simulink model "sim_taes_2023_att"  (R2020a)
settings: Solver=ode4  StartTime=0.0  StopTime=30.0  FixedStep=0.01  RelTol=1e-3
values from neighbouring files (symbols this model uses):
  c1_diff_sigma_bar_w = diag([12; 12; 12])    [init_taes_2023_att.m]
  c1_diff_ui = diag([25; 30; 20])    [init_taes_2023_att.m]
  c2_diff_sigma_bar_w = diag([12; 12; 12])    [init_taes_2023_att.m]
  c2_diff_ui = diag([50; 50; 10])    [init_taes_2023_att.m]
  c3_diff_sigma_bar_w = diag([15; 15; 15])    [init_taes_2023_att.m]
  c3_diff_ui = diag([15; 15; 10])    [init_taes_2023_att.m]
  cw = diag([4.0; 4.0; 4.0])    [init_taes_2023_att.m]
  dw_aa_t = 0.2 * ones(3, 5) + ( 1.0 - 0.2 ) * rand(3, 5)    [init_taes_2023_att.m]
  dw_ff_t = [ 0.4 * ones(1, 5) + ( 1.0 - 0.4 ) * rand(1, 5);                      0.4 * ones(1, 5) + ( 1.0 - 0.4 ) * rand(1, 5);                      0.2 * ones(1, 5) + ( 0.6 - 0.2 ) * rand(1, 5) ]    [init_taes_2023_att.m]
  dw_phi_t = ( - pi / 2 ) * ones(3, 5) + ( pi / 2 - ( - pi / 2 ) ) * rand(3, 5)    [init_taes_2023_att.m]
  dwci_init = zeros(3,5)    [init_taes_2023_att.m]
  h1w = diag([20.0; 20.0; 20.0])    [init_taes_2023_att.m]
  h2w = diag([35.0; 35.0; 35.0])    [init_taes_2023_att.m]
  h3w = diag([30.0; 30.0; 30.0])    [init_taes_2023_att.m]
  Ji = zeros(3,3,NF)    [init_taes_2023_att.m]
  kR = diag([40; 40; 40])    [init_taes_2023_att.m]
  kRtilt = diag([90; 90; 90])    [init_taes_2023_att.m]
  Lamd_diff_sigma_bar_w = 0.5    [init_taes_2023_att.m]
  Lamd_diff_ui = 0.5    [init_taes_2023_att.m]
  mu_d_w = 100    [init_taes_2023_att.m]
  pos0 = zeros(3, 1)    [init_taes_2023_att.m]
  PZ0 = P0(3)    [init_taes_2023_att.m]
  PZ1 = 10    [init_taes_2023_att.m]
  Qci_init = repmat([1;0;0;0],1,NF)    [init_taes_2023_att.m]
  R0 = 4    [init_taes_2023_att.m]
  R1 = 8    [init_taes_2023_att.m]
  Rci_init = zeros(3,3,NF)    [init_taes_2023_att.m]
  Ri_init = zeros(3,3,NF)    [init_taes_2023_att.m]
  Rx2 = 10    [init_taes_2023_att.m]
  Ry2 = 6    [init_taes_2023_att.m]
  Rz2 = 4    [init_taes_2023_att.m]
  T0 = 0    [init_taes_2023_att.m]
  T1 = tseq1    (= 10)    [init_taes_2023_att.m]
  T2 = tseq1 + tseq12 + tseq2    (= 30)    [init_taes_2023_att.m]
  ui_init = zeros(3,NF)    [init_taes_2023_att.m]
  vel0 = zeros(3, 1)    [init_taes_2023_att.m]
  wci_init = zeros(3,5)    [init_taes_2023_att.m]
  zeta_diff_sigma_bar_w = 0.08    [init_taes_2023_att.m]
  zeta_diff_ui = 0.08    [init_taes_2023_att.m]
undefined symbols (not defined in the file or in its folder): cal_frac_squ, p_alfaw1, p_alfaw2, q_alfaw1, q_alfaw2, Qei_init, Qeitilt_init, Qi_init, Rei_init, Reitilt_init, V_Phi_Rei_init, V_Phi_Reitilt_init, wei_init, weitilt_init, wi_init
(part 1 of 4)
settings Model: Creator=zzy  LastModifiedBy=Hershey.A
settings DataIOCC: ReturnWorkspaceOutputs=off
settings DebuggingCC: ArithmeticOperatorsInVariantConditions=warning
settings SFSimCC: SimUseLocalCustomCode=off  CustomCodeUndefinedFunction=UseInterfaceOnly
settings RTWCC: RTWUseLocalCustomCode=off

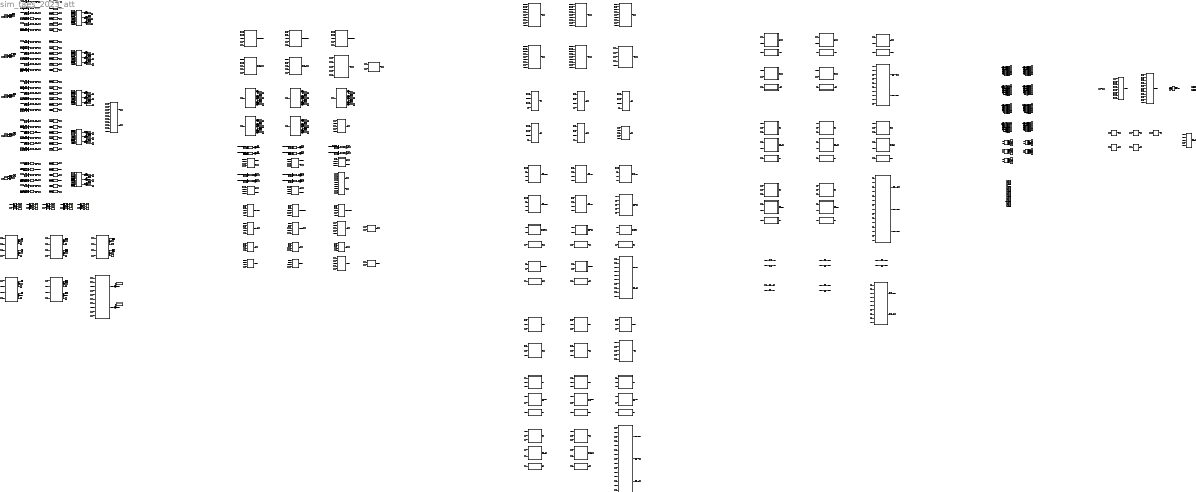
== system sim_taes_2023_att ==
  Abs{,1..29} (30 alike) : Abs
  Add{,1..2,4..6,8..10,12,14..16,18..19} (15 alike) : Sum
  Add{3,7,11,13,17} (5 alike) : Sum  Inputs=+-
  Clock : Clock
  Constant{,78,96,128,156} (5 alike) : Constant  Value=0
  Constant{1,3,5,7,9,46..47,49,65,67} (10 alike) : Constant  Value=h3w
  Constant{2,4,6,8,10,48,50,64,66,68,71,129..130,133,136,175..179} (20 alike) : Constant  Value=Ji
  Constant{51,54,59,61,63,79,82,87,89,91,97,100,105,107,109,114,119,121,123,139,142,147,149,151,157} (25 alike) : Constant
  Constant{52..53,55,62,74..75,80..81,83,90,92..93,98..99,101,108,110..111,115,122,124..125,140..141,143,150,152..153,158..159} (30 alike) : Constant  Value=3
  Constant{56,76,84,94,102,112,116,126,144,154} (10 alike) : Constant  Value=2
  Constant{57,85,103,117,145} (5 alike) : Constant  Value=c1_diff_ui
  Constant{58,86,104,118,146} (5 alike) : Constant  Value=c2_diff_ui
  Constant{60,88,106,120,148} (5 alike) : Constant  Value=c3_diff_ui
  Constant{11,13,18,23,28} (5 alike) : Constant  Value=p_alfaw1
  Constant{77,95,113,127,155} (5 alike) : Constant  Value=Lamd_diff_ui
  Constant{12,14,19,24,29} (5 alike) : Constant  Value=mu_d_w
  Constant{69,72,131,134,137} (5 alike) : Constant  Value=kR
  Constant{70,73,132,135,138} (5 alike) : Constant  Value=kRtilt
  Constant{15,20,25,30,33} (5 alike) : Constant  Value=q_alfaw1
  Constant{16,21,26,31,34} (5 alike) : Constant  Value=p_alfaw2
  Constant{160..174} (15 alike) : Constant  Value=zeta_diff_ui
  Constant{17,22,27,32,35} (5 alike) : Constant  Value=q_alfaw2
  Constant{180..184} (5 alike) : Constant  Value=cw
  Constant185 : Constant  Value=T1
  Constant186 : Constant  Value=R0
  Constant187 : Constant  Value=R1
  Constant188 : Constant  Value=T0
  Constant189 : Constant  Value=Rz2
  Constant190 : Constant  Value=Ry2
  Constant191 : Constant  Value=Rx2
  Constant192 : Constant  Value=T2
  Constant193 : Constant  Value=R0
  Constant194 : Constant  Value=R1
  Constant195 : Constant  Value=Rx2
  Constant196 : Constant  Value=Ry2
  Constant197 : Constant  Value=Rz2
  Constant198 : Constant  Value=T2
  Constant199 : Constant  Value=T1
  Constant200 : Constant  Value=PZ0
  Constant201 : Constant  Value=PZ1
  Constant{36,38,40,42,44} (5 alike) : Constant  Value=h1w
  Constant{37,39,41,43,45} (5 alike) : Constant  Value=h2w
  Constant{557,561,564,567,570} (5 alike) : Constant  Value=dw_aa_t
  Constant{558,562,565,568,572} (5 alike) : Constant  Value=dw_ff_t
  Constant{559,563,566,569,573} (5 alike) : Constant  Value=dw_phi_t
  Demux{,1..20,22..32,42..56,62..96} (82 alike) : Demux  Outputs=3
  Demux{33..37,57..61,97..101} (15 alike) : Demux
  Display{1..53,59..107} (102 alike) : Display
  Integrator{1..20} (20 alike) : Integrator  InitialCondition=zeros(3,1)
  Integrator21 : Integrator  InitialCondition=wi_init(:,1)
  Integrator22 : Integrator  InitialCondition=wi_init(:,2)
  Integrator23 : Integrator  InitialCondition=wi_init(:,3)
  Integrator24 : Integrator  InitialCondition=wi_init(:,4)
  Integrator25 : Integrator  InitialCondition=wi_init(:,5)
  Integrator26 : Integrator  InitialCondition=Qi_init(:,1)
  Integrator27 : Integrator  InitialCondition=Qi_init(:,2)
  Integrator28 : Integrator  InitialCondition=Qi_init(:,3)
  Integrator29 : Integrator  InitialCondition=Qi_init(:,4)
  Integrator30 : Integrator  InitialCondition=Qi_init(:,5)
  Integrator31 : Integrator  InitialCondition=Qei_init(:,1)
  Integrator32 : Integrator  InitialCondition=Qei_init(:,2)
  Integrator33 : Integrator  InitialCondition=Qei_init(:,3)
  Integrator34 : Integrator  InitialCondition=Qei_init(:,4)
  Integrator35 : Integrator  InitialCondition=Qei_init(:,5)
  Integrator36 : Integrator  InitialCondition=Qeitilt_init(:,1)
  Integrator37 : Integrator  InitialCondition=Qeitilt_init(:,2)
  Integrator38 : Integrator  InitialCondition=Qeitilt_init(:,3)
  Integrator39 : Integrator  InitialCondition=Qeitilt_init(:,4)
  Integrator40 : Integrator  InitialCondition=Qeitilt_init(:,5)
  Integrator41 : Integrator  InitialCondition=V_Phi_Reitilt_init(:,1)
  Integrator42 : Integrator  InitialCondition=V_Phi_Rei_init(:,2)
  Integrator43 : Integrator  InitialCondition=V_Phi_Reitilt_init(:,2)
  Integrator44 : Integrator  InitialCondition=V_Phi_Rei_init(:,3)
  Integrator45 : Integrator  InitialCondition=V_Phi_Rei_init(:,1)
  Integrator46 : Integrator  InitialCondition=V_Phi_Reitilt_init(:,3)
  Integrator47 : Integrator  InitialCondition=V_Phi_Rei_init(:,4)
  Integrator48 : Integrator  InitialCondition=V_Phi_Reitilt_init(:,4)
  Integrator49 : Integrator  InitialCondition=V_Phi_Rei_init(:,5)
  Integrator50 : Integrator  InitialCondition=V_Phi_Reitilt_init(:,5)
  Interpreted MATLAB Function{,1..39} (40 alike) : MATLABFcn  MATLABFcn=cal_frac_squ(u(1:3),u(4),u(5))
  Memory : Memory  InitialCondition=ui_init
  Memory10 : Memory  InitialCondition=Qeitilt_init
  Memory11 : Memory  InitialCondition=Reitilt_init
  Memory12 : Memory  InitialCondition=V_Phi_Rei_init
  Memory13 : Memory  InitialCondition=V_Phi_Reitilt_init
  Memory14 : Memory  InitialCondition=wci_init
  Memory15 : Memory  InitialCondition=dwci_init
  Memory16 : Memory  InitialCondition=Qci_init
  Memory17 : Memory  InitialCondition=Rci_init
  Memory3 : Memory  InitialCondition=Qi_init
  Memory4 : Memory  InitialCondition=Ri_init
  Memory5 : Memory  InitialCondition=wi_init
  Memory6 : Memory  InitialCondition=wei_init
  Memory7 : Memory  InitialCondition=Qei_init
  Memory8 : Memory  InitialCondition=Rei_init
  Memory9 : Memory  InitialCondition=weitilt_init
  Mux{,41..69} (30 alike) : Mux  Inputs=2
  Mux{1..40} (40 alike) : Mux  Inputs=3
  Product{,1..9} (10 alike) : Product
  Qei dynam agent 1 : MATLAB Function  TreatAsAtomicUnit=on
  Qei dynam agent 2 : MATLAB Function  TreatAsAtomicUnit=on
  Qei dynam agent 3 : MATLAB Function  TreatAsAtomicUnit=on
  Qei dynam agent 4 : MATLAB Function  TreatAsAtomicUnit=on
  Qei dynam agent 5 : MATLAB Function  TreatAsAtomicUnit=on
  Qeitilt dynam agent 1 : MATLAB Function  TreatAsAtomicUnit=on
  Qeitilt dynam agent 2 : MATLAB Function  TreatAsAtomicUnit=on
  Qeitilt dynam agent 3 : MATLAB Function  TreatAsAtomicUnit=on
  Qeitilt dynam agent 4 : MATLAB Function  TreatAsAtomicUnit=on
  Qeitilt dynam agent 5 : MATLAB Function  TreatAsAtomicUnit=on
  Qi dynam agent 1 : MATLAB Function  TreatAsAtomicUnit=on
  Qi dynam agent 2 : MATLAB Function  TreatAsAtomicUnit=on
  Qi dynam agent 3 : MATLAB Function  TreatAsAtomicUnit=on
  Qi dynam agent 4 : MATLAB Function  TreatAsAtomicUnit=on
  Qi dynam agent 5 : MATLAB Function  TreatAsAtomicUnit=on
  Scope{,3..11,45..49} (15 alike) : Scope  NumInputPorts=4
  Scope{1..2,12..44} (35 alike) : Scope  NumInputPorts=3
  Step : Step  Time=T1+0.01  SampleTime=0
  To Workspace : ToWorkspace  VariableName=wci  SampleTime=-1
  To Workspace1 : ToWorkspace  VariableName=V_Phi_Rei  SampleTime=-1
  To Workspace10 : ToWorkspace  VariableName=dwi_tilt  SampleTime=-1
  To Workspace11 : ToWorkspace  VariableName=Qci  SampleTime=-1
  To Workspace12 : ToWorkspace  VariableName=sigma_bar_w_hat  SampleTime=-1
  To Workspace13 : ToWorkspace  VariableName=wei  SampleTime=-1
  To Workspace14 : ToWorkspace  VariableName=sigma_w  SampleTime=-1
  To Workspace15 : ToWorkspace  VariableName=sigma_bar_w  SampleTime=-1
  To Workspace16 : ToWorkspace  VariableName=weitilt  SampleTime=-1
  To Workspace19 : ToWorkspace  VariableName=Qei  SampleTime=-1
  To Workspace2 : ToWorkspace  VariableName=wi  SampleTime=-1
  To Workspace20 : ToWorkspace  VariableName=Qi  SampleTime=-1
  To Workspace6 : ToWorkspace  VariableName=V_Phi_Reitilt  SampleTime=-1
  To Workspace7 : ToWorkspace  VariableName=Qeitilt  SampleTime=-1
  To Workspace8 : ToWorkspace  VariableName=dwi  SampleTime=-1
  To Workspace9 : ToWorkspace  VariableName=dwi_hat  SampleTime=-1
  cal Qci agent 1 : MATLAB Function  TreatAsAtomicUnit=on
  cal Qci agent 2 : MATLAB Function  TreatAsAtomicUnit=on
  cal Qci agent 3 : MATLAB Function  TreatAsAtomicUnit=on
  cal Qci agent 4 : MATLAB Function  TreatAsAtomicUnit=on
  cal Qci agent 5 : MATLAB Function  TreatAsAtomicUnit=on
  cal Rci agent 1 : MATLAB Function  TreatAsAtomicUnit=on
  cal Rci agent 2 : MATLAB Function  TreatAsAtomicUnit=on
  cal Rci agent 3 : MATLAB Function  TreatAsAtomicUnit=on
  cal Rci agent 4 : MATLAB Function  TreatAsAtomicUnit=on
  cal Rci agent 5 : MATLAB Function  TreatAsAtomicUnit=on
  cal Rei agent 1 : MATLAB Function  TreatAsAtomicUnit=on
  cal Rei agent 2 : MATLAB Function  TreatAsAtomicUnit=on
  cal Rei agent 3 : MATLAB Function  TreatAsAtomicUnit=on
  cal Rei agent 4 : MATLAB Function  TreatAsAtomicUnit=on
  cal Rei agent 5 : MATLAB Function  TreatAsAtomicUnit=on
  cal Reitilt agent 1 : MATLAB Function  TreatAsAtomicUnit=on
  cal Reitilt agent 2 : MATLAB Function  TreatAsAtomicUnit=on
  cal Reitilt agent 3 : MATLAB Function  TreatAsAtomicUnit=on
  cal Reitilt agent 4 : MATLAB Function  TreatAsAtomicUnit=on
  cal Reitilt agent 5 : MATLAB Function  TreatAsAtomicUnit=on
  cal Ri agent 1 : MATLAB Function  TreatAsAtomicUnit=on
  cal Ri agent 2 : MATLAB Function  TreatAsAtomicUnit=on
  cal Ri agent 3 : MATLAB Function  TreatAsAtomicUnit=on
  cal Ri agent 4 : MATLAB Function  TreatAsAtomicUnit=on
  cal Ri agent 5 : MATLAB Function  TreatAsAtomicUnit=on
  cal abs 21 : MATLAB Function  TreatAsAtomicUnit=on
  cal abs 22 : MATLAB Function  TreatAsAtomicUnit=on
  cal abs 23 : MATLAB Function  TreatAsAtomicUnit=on
  cal abs 24 : MATLAB Function  TreatAsAtomicUnit=on
  cal abs 25 : MATLAB Function  TreatAsAtomicUnit=on
  cal abs 26 : MATLAB Function  TreatAsAtomicUnit=on
  cal abs 27 : MATLAB Function  TreatAsAtomicUnit=on
  cal abs 28 : MATLAB Function  TreatAsAtomicUnit=on
  cal abs 29 : MATLAB Function  TreatAsAtomicUnit=on
  cal abs 30 : MATLAB Function  TreatAsAtomicUnit=on
  cal combine sigma_bar_w_tilt : MATLAB Function  TreatAsAtomicUnit=on
  cal d_sigma_w agent 1 : MATLAB Function  TreatAsAtomicUnit=on
  cal d_sigma_w agent 2 : MATLAB Function  TreatAsAtomicUnit=on
  cal d_sigma_w agent 3 : MATLAB Function  TreatAsAtomicUnit=on
  cal d_sigma_w agent 4 : MATLAB Function  TreatAsAtomicUnit=on
  cal d_sigma_w agent 5 : MATLAB Function  TreatAsAtomicUnit=on
  cal d_theta_hat : MATLAB Function  TreatAsAtomicUnit=on
  cal d_theta_hat1 : MATLAB Function  TreatAsAtomicUnit=on
  cal d_theta_hat2 : MATLAB Function  TreatAsAtomicUnit=on
  cal d_theta_hat3 : MATLAB Function  TreatAsAtomicUnit=on
  cal d_theta_hat4 : MATLAB Function  TreatAsAtomicUnit=on
  cal differentiator d_sigma_bar_w_hat agent 1 : Subsystem
  cal differentiator d_sigma_bar_w_hat agent 2 : Subsystem
  cal differentiator d_sigma_bar_w_hat agent 3 : Subsystem
  cal differentiator d_sigma_bar_w_hat agent 4 : Subsystem
  cal differentiator d_sigma_bar_w_hat agent 5 : Subsystem
  cal dw_hat agent 1 : MATLAB Function  TreatAsAtomicUnit=on
  cal dw_hat agent 2 : MATLAB Function  TreatAsAtomicUnit=on
  cal dw_hat agent 3 : MATLAB Function  TreatAsAtomicUnit=on
  cal dw_hat agent 4 : MATLAB Function  TreatAsAtomicUnit=on
  cal dw_hat agent 5 : MATLAB Function  TreatAsAtomicUnit=on
  cal error dw_tilt : MATLAB Function  TreatAsAtomicUnit=on
  cal sig : MATLAB Function  TreatAsAtomicUnit=on
  cal sig1 : MATLAB Function  TreatAsAtomicUnit=on
  cal sig10 : MATLAB Function  TreatAsAtomicUnit=on
  cal sig11 : MATLAB Function  TreatAsAtomicUnit=on
  cal sig12 : MATLAB Function  TreatAsAtomicUnit=on
  cal sig13 : MATLAB Function  TreatAsAtomicUnit=on
  cal sig14 : MATLAB Function  TreatAsAtomicUnit=on
  cal sig15 : MATLAB Function  TreatAsAtomicUnit=on
  cal sig16 : MATLAB Function  TreatAsAtomicUnit=on
  cal sig17 : MATLAB Function  TreatAsAtomicUnit=on
  cal sig18 : MATLAB Function  TreatAsAtomicUnit=on
  cal sig19 : MATLAB Function  TreatAsAtomicUnit=on
  cal sig2 : MATLAB Function  TreatAsAtomicUnit=on
  cal sig20 : MATLAB Function  TreatAsAtomicUnit=on
  cal sig21 : MATLAB Function  TreatAsAtomicUnit=on
  cal sig22 : MATLAB Function  TreatAsAtomicUnit=on
  cal sig23 : MATLAB Function  TreatAsAtomicUnit=on
  cal sig24 : MATLAB Function  TreatAsAtomicUnit=on
  cal sig25 : MATLAB Function  TreatAsAtomicUnit=on
  cal sig26 : MATLAB Function  TreatAsAtomicUnit=on
  cal sig27 : MATLAB Function  TreatAsAtomicUnit=on
  cal sig28 : MATLAB Function  TreatAsAtomicUnit=on
  cal sig29 : MATLAB Function  TreatAsAtomicUnit=on
  cal sig3 : MATLAB Function  TreatAsAtomicUnit=on
  cal sig4 : MATLAB Function  TreatAsAtomicUnit=on
  cal sig5 : MATLAB Function  TreatAsAtomicUnit=on
  cal sig6 : MATLAB Function  TreatAsAtomicUnit=on
  cal sig7 : MATLAB Function  TreatAsAtomicUnit=on
  cal sig8 : MATLAB Function  TreatAsAtomicUnit=on
  cal sig9 : MATLAB Function  TreatAsAtomicUnit=on
  cal sigma_bar_w_hat agent 1 : MATLAB Function  TreatAsAtomicUnit=on
  cal sigma_bar_w_hat agent 2 : MATLAB Function  TreatAsAtomicUnit=on
  cal sigma_bar_w_hat agent 3 : MATLAB Function  TreatAsAtomicUnit=on
  cal sigma_bar_w_hat agent 4 : MATLAB Function  TreatAsAtomicUnit=on
  cal sigma_bar_w_hat agent 5 : MATLAB Function  TreatAsAtomicUnit=on
  cal sigma_w_bar : MATLAB Function  TreatAsAtomicUnit=on
  cal taui agent 1 : MATLAB Function  TreatAsAtomicUnit=on
  cal taui agent 2 : MATLAB Function  TreatAsAtomicUnit=on
  cal taui agent 3 : MATLAB Function  TreatAsAtomicUnit=on
  cal taui agent 4 : MATLAB Function  TreatAsAtomicUnit=on
  cal taui agent 5 : MATLAB Function  TreatAsAtomicUnit=on
  cal theta_sigma_bar_w_tilt agent 1 : MATLAB Function  TreatAsAtomicUnit=on
  cal theta_sigma_bar_w_tilt agent 2 : MATLAB Function  TreatAsAtomicUnit=on
  cal theta_sigma_bar_w_tilt agent 3 : MATLAB Function  TreatAsAtomicUnit=on
  cal theta_sigma_bar_w_tilt agent 4 : MATLAB Function  TreatAsAtomicUnit=on
  cal theta_sigma_bar_w_tilt agent 5 : MATLAB Function  TreatAsAtomicUnit=on
  cal wbarei agent 1 : MATLAB Function  TreatAsAtomicUnit=on
  cal wbarei agent 2 : MATLAB Function  TreatAsAtomicUnit=on
  cal wbarei agent 3 : MATLAB Function  TreatAsAtomicUnit=on
  cal wbarei agent 4 : MATLAB Function  TreatAsAtomicUnit=on
  cal wbarei agent 5 : MATLAB Function  TreatAsAtomicUnit=on
  cal wci dwci agent 1 : MATLAB Function  TreatAsAtomicUnit=on
  cal wci dwci agent 2 : MATLAB Function  TreatAsAtomicUnit=on
  cal wci dwci agent 3 : MATLAB Function  TreatAsAtomicUnit=on
  cal wci dwci agent 4 : MATLAB Function  TreatAsAtomicUnit=on
  cal wci dwci agent 5 : MATLAB Function  TreatAsAtomicUnit=on
  cal wei agent 1 : MATLAB Function  TreatAsAtomicUnit=on
  cal wei agent 2 : MATLAB Function  TreatAsAtomicUnit=on
  cal wei agent 3 : MATLAB Function  TreatAsAtomicUnit=on
  cal wei agent 4 : MATLAB Function  TreatAsAtomicUnit=on
  cal wei agent 5 : MATLAB Function  TreatAsAtomicUnit=on
  cal weitilt agent 1 : MATLAB Function  TreatAsAtomicUnit=on
  cal weitilt agent 2 : MATLAB Function  TreatAsAtomicUnit=on
  cal weitilt agent 3 : MATLAB Function  TreatAsAtomicUnit=on
  cal weitilt agent 4 : MATLAB Function  TreatAsAtomicUnit=on
  cal weitilt agent 5 : MATLAB Function  TreatAsAtomicUnit=on
  choose ksi_est_err 21 : MATLAB Function  TreatAsAtomicUnit=on
  choose ksi_est_err 22 : MATLAB Function  TreatAsAtomicUnit=on
  choose ksi_est_err 23 : MATLAB Function  TreatAsAtomicUnit=on
  choose ksi_est_err 24 : MATLAB Function  TreatAsAtomicUnit=on
  choose ksi_est_err 25 : MATLAB Function  TreatAsAtomicUnit=on
  choose ksi_est_err 26 : MATLAB Function  TreatAsAtomicUnit=on
  choose ksi_est_err 27 : MATLAB Function  TreatAsAtomicUnit=on
  choose ksi_est_err 28 : MATLAB Function  TreatAsAtomicUnit=on
  choose ksi_est_err 29 : MATLAB Function  TreatAsAtomicUnit=on
  choose ksi_est_err 30 : MATLAB Function  TreatAsAtomicUnit=on
  choose ui agent 1 : MATLAB Function  TreatAsAtomicUnit=on
  choose ui agent 2 : MATLAB Function  TreatAsAtomicUnit=on
  choose ui agent 3 : MATLAB Function  TreatAsAtomicUnit=on
  choose ui agent 4 : MATLAB Function  TreatAsAtomicUnit=on
  choose ui agent 5 : MATLAB Function  TreatAsAtomicUnit=on
  combine Qci Rci : MATLAB Function  TreatAsAtomicUnit=on
  combine Qci Rci1 : MATLAB Function  TreatAsAtomicUnit=on
  combine Qi Ri : MATLAB Function  TreatAsAtomicUnit=on
  combine d_sigma_bar_v_est : MATLAB Function  TreatAsAtomicUnit=on
  combine duihat d2uihat : MATLAB Function  TreatAsAtomicUnit=on
  combine dw_hat : MATLAB Function  TreatAsAtomicUnit=on
  combine dwi : MATLAB Function  TreatAsAtomicUnit=on
  combine norminal formation control input : MATLAB Function  TreatAsAtomicUnit=on
  combine sigma_bar_w_hat : MATLAB Function  TreatAsAtomicUnit=on
  combine sigma_w : MATLAB Function  TreatAsAtomicUnit=on
  combine tau : MATLAB Function  TreatAsAtomicUnit=on
  combine tau1 : MATLAB Function  TreatAsAtomicUnit=on
  combine theta_sigma_bar_w_tilt : MATLAB Function  TreatAsAtomicUnit=on
  combine wbarei : MATLAB Function  TreatAsAtomicUnit=on
  combine wci dwci : MATLAB Function  TreatAsAtomicUnit=on
  combine wei Qei Rei : MATLAB Function  TreatAsAtomicUnit=on
  combine weitilt Qeitilt Reitilt : MATLAB Function  TreatAsAtomicUnit=on
  control input generator agent 1 : MATLAB Function  TreatAsAtomicUnit=on
  control input generator agent 2 : MATLAB Function  TreatAsAtomicUnit=on
  control input generator agent 3 : MATLAB Function  TreatAsAtomicUnit=on
  control input generator agent 4 : MATLAB Function  TreatAsAtomicUnit=on
  control input generator agent 5 : MATLAB Function  TreatAsAtomicUnit=on
  d2_sigma_bar_w_est_{1..5} (5 alike) : Scope  NumInputPorts=3
  d2_ui_hat_node_{1..5} (5 alike) : Scope  NumInputPorts=3
  d_sigma_bar_w_est_{1..5} (5 alike) : Scope  NumInputPorts=3
  d_ui_hat_node_{1..5} (5 alike) : Scope  NumInputPorts=3
  depart Qc1 : MATLAB Function  TreatAsAtomicUnit=on
  depart Qc2 : MATLAB Function  TreatAsAtomicUnit=on
  depart Qc3 : MATLAB Function  TreatAsAtomicUnit=on
  depart Qc4 : MATLAB Function  TreatAsAtomicUnit=on
  depart Qc5 : MATLAB Function  TreatAsAtomicUnit=on
  depart Qe1 : MATLAB Function  TreatAsAtomicUnit=on
  depart Qe1tilt : MATLAB Function  TreatAsAtomicUnit=on
  depart Qe2 : MATLAB Function  TreatAsAtomicUnit=on
  depart Qe2tilt : MATLAB Function  TreatAsAtomicUnit=on
  depart Qe3 : MATLAB Function  TreatAsAtomicUnit=on
  depart Qe3tilt : MATLAB Function  TreatAsAtomicUnit=on
  depart Qe4 : MATLAB Function  TreatAsAtomicUnit=on
  depart Qe4tilt : MATLAB Function  TreatAsAtomicUnit=on
  depart Qe5 : MATLAB Function  TreatAsAtomicUnit=on
  depart Qe5tilt : MATLAB Function  TreatAsAtomicUnit=on
  depart V_Phi_Re1 : MATLAB Function  TreatAsAtomicUnit=on
  depart V_Phi_Re1tilt : MATLAB Function  TreatAsAtomicUnit=on
  depart V_Phi_Re2 : MATLAB Function  TreatAsAtomicUnit=on
  depart V_Phi_Re2tilt : MATLAB Function  TreatAsAtomicUnit=on
  depart V_Phi_Re3 : MATLAB Function  TreatAsAtomicUnit=on
  depart V_Phi_Re3tilt : MATLAB Function  TreatAsAtomicUnit=on
  depart V_Phi_Re4 : MATLAB Function  TreatAsAtomicUnit=on
  depart V_Phi_Re4tilt : MATLAB Function  TreatAsAtomicUnit=on
  depart V_Phi_Re5 : MATLAB Function  TreatAsAtomicUnit=on
  depart V_Phi_Re5tilt : MATLAB Function  TreatAsAtomicUnit=on
  depart dw1 dw_hat_1 : MATLAB Function  TreatAsAtomicUnit=on
  depart dw2 dw_hat_2 : MATLAB Function  TreatAsAtomicUnit=on
  depart dw3 dw_hat_3 : MATLAB Function  TreatAsAtomicUnit=on
  depart dw4 dw_hat_1 : MATLAB Function  TreatAsAtomicUnit=on
  depart dw4 dw_hat_4 : MATLAB Function  TreatAsAtomicUnit=on
  depart wc1 : MATLAB Function  TreatAsAtomicUnit=on
  depart wc2 : MATLAB Function  TreatAsAtomicUnit=on
  depart wc3 : MATLAB Function  TreatAsAtomicUnit=on
  depart wc4 : MATLAB Function  TreatAsAtomicUnit=on
  depart wc5 : MATLAB Function  TreatAsAtomicUnit=on
  depart we1 : MATLAB Function  TreatAsAtomicUnit=on
  depart we1tilt : MATLAB Function  TreatAsAtomicUnit=on
  depart we2 : MATLAB Function  TreatAsAtomicUnit=on
  depart we2tilt : MATLAB Function  TreatAsAtomicUnit=on
  depart we3 : MATLAB Function  TreatAsAtomicUnit=on
  depart we3tilt : MATLAB Function  TreatAsAtomicUnit=on
  depart we4 : MATLAB Function  TreatAsAtomicUnit=on
  depart we4tilt : MATLAB Function  TreatAsAtomicUnit=on
  depart we5 : MATLAB Function  TreatAsAtomicUnit=on
  depart we5tilt : MATLAB Function  TreatAsAtomicUnit=on
  dwci_node_{1..5} (5 alike) : Scope  NumInputPorts=3
  eta_0 : Scope  NumInputPorts=3
  generate angular rate disturbance agent 1 : MATLAB Function  TreatAsAtomicUnit=on
  generate angular rate disturbance agent 2 : MATLAB Function  TreatAsAtomicUnit=on
  generate angular rate disturbance agent 3 : MATLAB Function  TreatAsAtomicUnit=on
  generate angular rate disturbance agent 4 : MATLAB Function  TreatAsAtomicUnit=on
  generate angular rate disturbance agent 5 : MATLAB Function  TreatAsAtomicUnit=on
  ksi_0 : Scope  NumInputPorts=3
  leader control input : MATLAB Function  TreatAsAtomicUnit=on
  leader eta0 Integrator : Integrator  ExternalReset=rising  InitialConditionSource=external  InitialCondition=vel0
  leader ksi0 Integrator : Integrator  InitialCondition=pos0
  process velocity : MATLAB Function  TreatAsAtomicUnit=on
  sigma_bar_w_hat Integrator {1..5} (5 alike) : Integrator  InitialCondition=zeros(3,1)
  trans to column1 : MATLAB Function  TreatAsAtomicUnit=on
  trans to column10 : MATLAB Function  TreatAsAtomicUnit=on
  trans to column11 : MATLAB Function  TreatAsAtomicUnit=on
  trans to column12 : MATLAB Function  TreatAsAtomicUnit=on
  trans to column13 : MATLAB Function  TreatAsAtomicUnit=on
  trans to column14 : MATLAB Function  TreatAsAtomicUnit=on
  trans to column15 : MATLAB Function  TreatAsAtomicUnit=on
  trans to column16 : MATLAB Function  TreatAsAtomicUnit=on
  trans to column17 : MATLAB Function  TreatAsAtomicUnit=on
  trans to column18 : MATLAB Function  TreatAsAtomicUnit=on
  trans to column19 : MATLAB Function  TreatAsAtomicUnit=on
  trans to column2 : MATLAB Function  TreatAsAtomicUnit=on
  trans to column20 : MATLAB Function  TreatAsAtomicUnit=on
  trans to column21 : MATLAB Function  TreatAsAtomicUnit=on
  trans to column22 : MATLAB Function  TreatAsAtomicUnit=on
  trans to column23 : MATLAB Function  TreatAsAtomicUnit=on
  trans to column24 : MATLAB Function  TreatAsAtomicUnit=on
  trans to column25 : MATLAB Function  TreatAsAtomicUnit=on
  trans to column26 : MATLAB Function  TreatAsAtomicUnit=on
  trans to column27 : MATLAB Function  TreatAsAtomicUnit=on
  trans to column28 : MATLAB Function  TreatAsAtomicUnit=on
  trans to column29 : MATLAB Function  TreatAsAtomicUnit=on
  trans to column3 : MATLAB Function  TreatAsAtomicUnit=on
  trans to column30 : MATLAB Function  TreatAsAtomicUnit=on
  trans to column31 : MATLAB Function  TreatAsAtomicUnit=on
  trans to column32 : MATLAB Function  TreatAsAtomicUnit=on
  trans to column33 : MATLAB Function  TreatAsAtomicUnit=on
  trans to column34 : MATLAB Function  TreatAsAtomicUnit=on
  trans to column35 : MATLAB Function  TreatAsAtomicUnit=on
  trans to column36 : MATLAB Function  TreatAsAtomicUnit=on
  trans to column37 : MATLAB Function  TreatAsAtomicUnit=on
  trans to column38 : MATLAB Function  TreatAsAtomicUnit=on
  trans to column39 : MATLAB Function  TreatAsAtomicUnit=on
  trans to column4 : MATLAB Function  TreatAsAtomicUnit=on
  trans to column40 : MATLAB Function  TreatAsAtomicUnit=on
  trans to column5 : MATLAB Function  TreatAsAtomicUnit=on
  trans to column6 : MATLAB Function  TreatAsAtomicUnit=on
  trans to column7 : MATLAB Function  TreatAsAtomicUnit=on
  trans to column8 : MATLAB Function  TreatAsAtomicUnit=on
  trans to column9 : MATLAB Function  TreatAsAtomicUnit=on
  ui_tilt_node_{1..5} (5 alike) : Scope  NumInputPorts=3
  wci_node_{1..5} (5 alike) : Scope  NumInputPorts=3
  wi dynam agent 1 : MATLAB Function  TreatAsAtomicUnit=on
  wi dynam agent 2 : MATLAB Function  TreatAsAtomicUnit=on
  wi dynam agent 3 : MATLAB Function  TreatAsAtomicUnit=on
  wi dynam agent 4 : MATLAB Function  TreatAsAtomicUnit=on
  wi dynam agent 5 : MATLAB Function  TreatAsAtomicUnit=on
  wires:
  [d_ui_hat_node_1] -> cal d_theta_hat/11(dui_hat)
  [ui_sig_3_node_1] -> cal d_theta_hat/7(ui_sig_3)
  cal d_theta_hat/2(d_dui_hat) -> Integrator3/1
  Constant63/1 -> Mux8/2
  Mux10/1 -> Interpreted MATLAB Function9/1
  cal sig5/1(z) -> [ui_sig_5_node_1]
  Interpreted MATLAB Function8/1 -> trans to column8/1(x)
  Interpreted MATLAB Function9/1 -> trans to column9/1(x)
  [ui_squ_3_node_1] -> cal sig2/1(x)
  Constant163/1 -> Product1/2
  [ui_squ_6_node_1] -> cal sig3/1(x)
  [ui_sig_6_node_1] -> cal d_theta_hat/10(ui_sig_6)
  cal d_theta_hat/3(d_d2ui_hat) -> Integrator4/1
  trans to column8/1(y) -> [ui_squ_4_node_1]
  [ui_tilt_node_1] -> cal sig1/2(y)
  [ui_sig_2_node_1] -> cal d_theta_hat/6(ui_sig_2)
  Abs/1 -> Mux7/1
  Constant56/1 -> Mux11/2
  [d2_ui_hat_node_1] -> cal d_theta_hat/12(d2ui_hat)
  cal sig3/1(z) -> [ui_sig_6_node_1]
  Interpreted MATLAB Function7/1 -> trans to column7/1(x)
  Interpreted MATLAB Function/1 -> trans to column6/1(x)
  cal sig4/1(z) -> [ui_sig_4_node_1]
  Product1/1 -> Add2/2
  [ui_tilt_node_1] -> cal sig5/2(y)
  trans to column10/1(y) -> [ui_squ_5_node_1]
  [ui_tilt_node_1] -> cal sig/2(y)
  Interpreted MATLAB Function10/1 -> trans to column10/1(x)
  Mux11/1 -> Interpreted MATLAB Function10/1
  Abs5/1 -> Mux11/1
  Abs3/1 -> Mux9/1
  Constant53/1 -> Add2/1
  Constant/1 -> Mux7/2
  Constant162/1 -> Product/2
  Constant54/1 -> Product1/1
  Constant55/1 -> Mux11/3
  [ui_tilt_node_1] -> Abs4/1
  [ui_sig_4_node_1] -> cal d_theta_hat/8(ui_sig_4)
  [ui_sig_1_node_1] -> cal d_theta_hat/5(ui_sig_1)
  [ui_squ_5_node_1] -> cal sig5/1(x)
  Constant59/1 -> Add/1
  Constant61/1 -> Mux6/3
  Mux7/1 -> Interpreted MATLAB Function/1
  Mux8/1 -> Interpreted MATLAB Function7/1
  Constant161/1 -> Add/2
  [ui_tilt_node_1] -> Abs2/1
  [ui_tilt_node_1] -> Abs1/1
  [ui_tilt_node_1] -> Abs5/1
  Mux6/1 -> Interpreted MATLAB Function6/1
  Interpreted MATLAB Function6/1 -> trans to column5/1(x)
  Add/1 -> Mux6/2
  [ui_squ_4_node_1] -> cal sig4/1(x)
  trans to column9/1(y) -> [ui_squ_6_node_1]
  trans to column7/1(y) -> [ui_squ_3_node_1]
  [ui_tilt_node_1] -> cal sig4/2(y)
  [ui_tilt_node_1] -> cal sig3/2(y)
  Product/1 -> Add1/2
  Constant51/1 -> Mux7/3
  Constant75/1 -> Add1/1
  [ui_tilt_node_1] -> Abs/1
  [ui_tilt_node_1] -> Abs3/1
  Mux9/1 -> Interpreted MATLAB Function8/1
  Abs2/1 -> Mux8/1
  Constant62/1 -> Mux8/3
  trans to column5/1(y) -> [ui_squ_2_node_1]
  cal sig1/1(z) -> [ui_sig_2_node_1]
  Constant52/1 -> Mux10/3
  cal sig/1(z) -> [ui_sig_1_node_1]
  Abs4/1 -> Mux10/1
  cal sig2/1(z) -> [ui_sig_3_node_1]
  Abs1/1 -> Mux6/1
  Constant74/1 -> Mux9/3
  Add2/1 -> Mux10/2
  [ui_sig_5_node_1] -> cal d_theta_hat/9(ui_sig_5)
  Add1/1 -> Mux9/2
  Constant76/1 -> Product/1
  [ui_tilt_node_1] -> cal sig2/2(y)
  [ui_squ_2_node_1] -> cal sig1/1(x)
  [ui_squ_1_node_1] -> cal sig/1(x)
  trans to column6/1(y) -> [ui_squ_1_node_1]
  Constant57/1 -> cal d_theta_hat/1(c1)
  Constant58/1 -> cal d_theta_hat/2(c2)
  Constant60/1 -> cal d_theta_hat/3(c3)
  Constant77/1 -> cal d_theta_hat/4(chi_t)
  Integrator4/1 -> Display24/1, Demux12/1, [d2_ui_hat_node_1]
  cal d_theta_hat/1(d_ui_hat) -> Integrator2/1
  Integrator3/1 -> Demux8/1, Display23/1, [d_ui_hat_node_1]
  Integrator2/1 -> Display22/1, [ui_hat_node_1]
  [ui_hat_node_1] -> Add3/1
  Add3/1 -> Demux2/1, [ui_tilt_node_1]
  [ui_vec] -> choose ui agent 1/1(x)
  choose ui agent 1/1(y) -> Add3/2
  [ui_squ_1_node_2] -> cal sig6/1(x)
  [ui_squ_2_node_2] -> cal sig7/1(x)
  [ui_tilt_node_2] -> cal sig8/2(y)
  Constant94/1 -> Product2/1
  Constant95/1 -> cal d_theta_hat1/4(chi_t)
  Add7/1 -> Demux3/1, [ui_tilt_node_2]
  [ui_hat_node_2] -> Add7/1
  [ui_sig_5_node_2] -> cal d_theta_hat1/9(ui_sig_5)
  Add6/1 -> Mux12/2
  Add5/1 -> Mux17/2
  Constant92/1 -> Mux17/3
  Constant80/1 -> Mux12/3
  cal sig6/1(z) -> [ui_sig_1_node_2]
  trans to column12/1(y) -> [ui_squ_2_node_2]
  cal sig7/1(z) -> [ui_sig_2_node_2]
  cal sig8/1(z) -> [ui_sig_3_node_2]
  Abs7/1 -> Mux14/1
  Abs10/1 -> Mux12/1
  Constant90/1 -> Mux16/3
  [ui_tilt_node_2] -> Abs9/1
  Mux17/1 -> Interpreted MATLAB Function15/1
  choose ui agent 2/1(y) -> Add7/2
  Abs8/1 -> Mux16/1
  Product2/1 -> Add5/2
  [ui_tilt_node_2] -> Abs6/1
  Constant93/1 -> Add5/1
  [ui_tilt_node_2] -> cal sig10/2(y)
  Constant79/1 -> Mux15/3
  trans to column16/1(y) -> [ui_squ_6_node_2]
  Constant88/1 -> cal d_theta_hat1/3(c3)
  Constant85/1 -> cal d_theta_hat1/1(c1)
  Integrator1/1 -> Display25/1, [ui_hat_node_2]
  Integrator6/1 -> Display27/1, Demux13/1, [d2_ui_hat_node_2]
  trans to column15/1(y) -> [ui_squ_4_node_2]
  [ui_sig_6_node_2] -> cal d_theta_hat1/10(ui_sig_6)
  [ui_squ_6_node_2] -> cal sig9/1(x)
  Constant91/1 -> Mux16/2
  [ui_squ_4_node_2] -> cal sig10/1(x)
  [d_ui_hat_node_2] -> cal d_theta_hat1/11(dui_hat)
  Mux14/1 -> Interpreted MATLAB Function13/1
  [ui_tilt_node_2] -> cal sig9/2(y)
  Constant160/1 -> Add4/2
  Constant87/1 -> Add4/1
  Mux12/1 -> Interpreted MATLAB Function16/1
  [ui_squ_5_node_2] -> cal sig11/1(x)
  [ui_sig_1_node_2] -> cal d_theta_hat1/5(ui_sig_1)
  [ui_tilt_node_2] -> Abs8/1
  [ui_sig_4_node_2] -> cal d_theta_hat1/8(ui_sig_4)
  [ui_tilt_node_2] -> Abs10/1
  cal d_theta_hat1/2(d_dui_hat) -> Integrator5/1
  Constant89/1 -> Mux14/3
  Constant83/1 -> Mux13/3
  Constant82/1 -> Product3/1
  Abs9/1 -> Mux17/1
  Interpreted MATLAB Function11/1 -> trans to column13/1(x)
  Mux16/1 -> Interpreted MATLAB Function14/1
  trans to column13/1(y) -> [ui_squ_1_node_2]
  Interpreted MATLAB Function16/1 -> trans to column16/1(x)
  Interpreted MATLAB Function12/1 -> trans to column11/1(x)
  Constant81/1 -> Add6/1
  Abs11/1 -> Mux13/1
  cal sig10/1(z) -> [ui_sig_4_node_2]
  [ui_tilt_node_2] -> cal sig6/2(y)
  Constant78/1 -> Mux15/2
  Interpreted MATLAB Function14/1 -> trans to column14/1(x)
  Constant164/1 -> Product2/2
  [ui_vec] -> choose ui agent 2/1(x)
  [d2_ui_hat_node_2] -> cal d_theta_hat1/12(d2ui_hat)
  Add4/1 -> Mux14/2
  trans to column11/1(y) -> [ui_squ_5_node_2]
  cal d_theta_hat1/1(d_ui_hat) -> Integrator1/1
  Constant165/1 -> Product3/2
  cal sig9/1(z) -> [ui_sig_6_node_2]
  Abs6/1 -> Mux15/1
  [ui_tilt_node_2] -> Abs7/1
  Interpreted MATLAB Function15/1 -> trans to column15/1(x)
  cal d_theta_hat1/3(d_d2ui_hat) -> Integrator6/1
  [ui_sig_2_node_2] -> cal d_theta_hat1/6(ui_sig_2)
  Product3/1 -> Add6/2
  Mux15/1 -> Interpreted MATLAB Function11/1
  [ui_tilt_node_2] -> Abs11/1
  [ui_tilt_node_2] -> cal sig11/2(y)
  Interpreted MATLAB Function13/1 -> trans to column12/1(x)
  [ui_tilt_node_2] -> cal sig7/2(y)
  Constant84/1 -> Mux13/2
  Mux13/1 -> Interpreted MATLAB Function12/1
  [ui_sig_3_node_2] -> cal d_theta_hat1/7(ui_sig_3)
  trans to column14/1(y) -> [ui_squ_3_node_2]
  Constant86/1 -> cal d_theta_hat1/2(c2)
  cal sig11/1(z) -> [ui_sig_5_node_2]
  [ui_squ_3_node_2] -> cal sig8/1(x)
  [ui_squ_4_node_3] -> cal sig12/1(x)
  Constant109/1 -> Mux22/2
  [ui_squ_6_node_3] -> cal sig17/1(x)
  [ui_sig_6_node_3] -> cal d_theta_hat2/10(ui_sig_6)
  trans to column21/1(y) -> [ui_squ_4_node_3]
  Integrator9/1 -> Display30/1, Demux14/1, [d2_ui_hat_node_3]
  Integrator8/1 -> Display29/1, Demux7/1, [d_ui_hat_node_3]
  Integrator7/1 -> Display28/1, [ui_hat_node_3]
  Constant103/1 -> cal d_theta_hat2/1(c1)
  Constant106/1 -> cal d_theta_hat2/3(c3)
  [ui_tilt_node_3] -> Abs14/1
  trans to column22/1(y) -> [ui_squ_6_node_3]
  Constant97/1 -> Mux21/3
  Product4/1 -> Add9/2
  [ui_tilt_node_3] -> cal sig12/2(y)
  Constant111/1 -> Add9/1
  Abs12/1 -> Mux18/1
  cal sig16/1(z) -> [ui_sig_3_node_3]
  Constant108/1 -> Mux22/3
  [ui_tilt_node_3] -> Abs17/1
  Abs15/1 -> Mux20/1
  Abs16/1 -> Mux22/1
  choose ui agent 3/1(y) -> Add11/2
  Mux23/1 -> Interpreted MATLAB Function21/1
  cal sig15/1(z) -> [ui_sig_2_node_3]
  trans to column18/1(y) -> [ui_squ_2_node_3]
  cal sig14/1(z) -> [ui_sig_1_node_3]
  Constant98/1 -> Mux18/3
  Add11/1 -> Demux4/1, [ui_tilt_node_3]
  Constant113/1 -> cal d_theta_hat2/4(chi_t)
  Constant112/1 -> Product4/1
  Constant110/1 -> Mux23/3
  Add9/1 -> Mux23/2
  [ui_sig_5_node_3] -> cal d_theta_hat2/9(ui_sig_5)
  [ui_hat_node_3] -> Add11/1
  Add10/1 -> Mux18/2
  [ui_tilt_node_3] -> cal sig16/2(y)
  [ui_sig_1_node_3] -> cal d_theta_hat2/5(ui_sig_1)
  [ui_sig_4_node_3] -> cal d_theta_hat2/8(ui_sig_4)
  Mux18/1 -> Interpreted MATLAB Function22/1
  [ui_tilt_node_3] -> cal sig17/2(y)
  [ui_squ_5_node_3] -> cal sig13/1(x)
  Mux20/1 -> Interpreted MATLAB Function19/1
  Interpreted MATLAB Function18/1 -> trans to column17/1(x)
  [ui_tilt_node_3] -> Abs12/1
  Mux22/1 -> Interpreted MATLAB Function20/1
  Interpreted MATLAB Function17/1 -> trans to column19/1(x)
  Abs17/1 -> Mux23/1
  cal sig17/1(z) -> [ui_sig_6_node_3]
  Abs13/1 -> Mux19/1
  cal d_theta_hat2/1(d_ui_hat) -> Integrator7/1
  trans to column19/1(y) -> [ui_squ_1_node_3]
  trans to column17/1(y) -> [ui_squ_5_node_3]
  [d_ui_hat_node_3] -> cal d_theta_hat2/11(dui_hat)
  [d2_ui_hat_node_3] -> cal d_theta_hat2/12(d2ui_hat)
  Interpreted MATLAB Function22/1 -> trans to column22/1(x)
  Interpreted MATLAB Function20/1 -> trans to column20/1(x)
  cal d_theta_hat2/2(d_dui_hat) -> Integrator8/1
  Constant167/1 -> Product4/2
  Constant101/1 -> Mux19/3
  Constant105/1 -> Add8/1
  Constant96/1 -> Mux21/2
  [ui_tilt_node_3] -> cal sig14/2(y)
  cal sig12/1(z) -> [ui_sig_4_node_3]
  Constant168/1 -> Product5/2
  cal sig13/1(z) -> [ui_sig_5_node_3]
  [ui_squ_3_node_3] -> cal sig16/1(x)
  [ui_sig_3_node_3] -> cal d_theta_hat2/7(ui_sig_3)
  Mux19/1 -> Interpreted MATLAB Function18/1
  Constant104/1 -> cal d_theta_hat2/2(c2)
  Constant102/1 -> Mux19/2
  trans to column20/1(y) -> [ui_squ_3_node_3]
  [ui_tilt_node_3] -> Abs16/1
  Interpreted MATLAB Function19/1 -> trans to column18/1(x)
  [ui_tilt_node_3] -> cal sig15/2(y)
  Constant166/1 -> Add8/2
  [ui_tilt_node_3] -> Abs13/1
  [ui_tilt_node_3] -> cal sig13/2(y)
  [ui_squ_1_node_3] -> cal sig14/1(x)
  [ui_sig_2_node_3] -> cal d_theta_hat2/6(ui_sig_2)
  [ui_tilt_node_3] -> Abs15/1
  Interpreted MATLAB Function21/1 -> trans to column21/1(x)
  [ui_vec] -> choose ui agent 3/1(x)
  Constant99/1 -> Add10/1
  cal d_theta_hat2/3(d_d2ui_hat) -> Integrator9/1
  Abs14/1 -> Mux21/1
  Constant107/1 -> Mux20/3
  Product5/1 -> Add10/2
  [ui_squ_2_node_3] -> cal sig15/1(x)
  Add8/1 -> Mux20/2
  Constant100/1 -> Product5/1
  Mux21/1 -> Interpreted MATLAB Function17/1
  [ui_vec] -> choose ui agent 4/1(x)
  [ui_sig_2_node_4] -> cal d_theta_hat3/6(ui_sig_2)
  [ui_tilt_node_4] -> cal sig19/2(y)
  [ui_squ_1_node_4] -> cal sig20/1(x)
  [ui_tilt_node_4] -> Abs19/1
  trans to column26/1(y) -> [ui_squ_3_node_4]
  Constant169/1 -> Add14/2
  Interpreted MATLAB Function25/1 -> trans to column24/1(x)
  [ui_tilt_node_4] -> cal sig21/2(y)
  [ui_tilt_node_4] -> Abs22/1
  [ui_squ_3_node_4] -> cal sig22/1(x)
  [ui_sig_3_node_4] -> cal d_theta_hat3/7(ui_sig_3)
  Constant116/1 -> Mux25/2
  Mux25/1 -> Interpreted MATLAB Function24/1
  cal sig19/1(z) -> [ui_sig_5_node_4]
  Constant128/1 -> Mux27/2
  [ui_tilt_node_4] -> cal sig20/2(y)
  Constant171/1 -> Product7/2
  cal sig18/1(z) -> [ui_sig_4_node_4]
  Constant119/1 -> Add14/1
  Constant115/1 -> Mux25/3
  Constant170/1 -> Product6/2
  cal d_theta_hat3/2(d_dui_hat) -> Integrator11/1
  Interpreted MATLAB Function26/1 -> trans to column26/1(x)
  Interpreted MATLAB Function28/1 -> trans to column28/1(x)
  cal d_theta_hat3/1(d_ui_hat) -> Integrator10/1
  [d2_ui_hat_node_4] -> cal d_theta_hat3/12(d2ui_hat)
  [d_ui_hat_node_4] -> cal d_theta_hat3/11(dui_hat)
  trans to column23/1(y) -> [ui_squ_5_node_4]
  Constant118/1 -> cal d_theta_hat3/2(c2)
  Interpreted MATLAB Function24/1 -> trans to column23/1(x)
  Abs23/1 -> Mux29/1
  [ui_squ_5_node_4] -> cal sig19/1(x)
  [ui_tilt_node_4] -> Abs18/1
  [ui_tilt_node_4] -> cal sig23/2(y)
  Mux24/1 -> Interpreted MATLAB Function28/1
  Add15/1 -> Mux29/2
  Add12/1 -> Mux24/2
  Interpreted MATLAB Function23/1 -> trans to column25/1(x)
  Abs19/1 -> Mux25/1
  Constant124/1 -> Mux29/3
  trans to column24/1(y) -> [ui_squ_2_node_4]
  Constant140/1 -> Mux24/3
  Mux29/1 -> Interpreted MATLAB Function27/1
  cal sig21/1(z) -> [ui_sig_2_node_4]
  Abs21/1 -> Mux26/1
  Abs18/1 -> Mux24/1
  [ui_tilt_node_4] -> Abs23/1
  [ui_sig_5_node_4] -> cal d_theta_hat3/9(ui_sig_5)
  Constant122/1 -> Mux28/3
  Constant125/1 -> Add15/1
  cal sig22/1(z) -> [ui_sig_3_node_4]
  Abs22/1 -> Mux28/1
  [ui_tilt_node_4] -> cal sig18/2(y)
  Constant117/1 -> cal d_theta_hat3/1(c1)
  Constant120/1 -> cal d_theta_hat3/3(c3)
  cal sig20/1(z) -> [ui_sig_1_node_4]
  trans to column28/1(y) -> [ui_squ_6_node_4]
  Integrator10/1 -> [ui_hat_node_4], Display31/1
  [ui_tilt_node_4] -> Abs20/1
  Product6/1 -> Add15/2
  trans to column25/1(y) -> [ui_squ_1_node_4]
  [ui_squ_6_node_4] -> cal sig23/1(x)
  Integrator11/1 -> Display32/1, Demux10/1, [d_ui_hat_node_4]
  trans to column27/1(y) -> [ui_squ_4_node_4]
  [ui_hat_node_4] -> Add13/1
  Constant126/1 -> Product6/1
  Integrator12/1 -> Display33/1, Demux15/1, [d2_ui_hat_node_4]
  Constant139/1 -> Mux27/3
  [ui_squ_4_node_4] -> cal sig18/1(x)
  Constant127/1 -> cal d_theta_hat3/4(chi_t)
  Constant123/1 -> Mux28/2
  [ui_tilt_node_4] -> Abs21/1
  Interpreted MATLAB Function27/1 -> trans to column27/1(x)
  choose ui agent 4/1(y) -> Add13/2
  Add13/1 -> Demux5/1, [ui_tilt_node_4]
  [ui_sig_6_node_4] -> cal d_theta_hat3/10(ui_sig_6)
  [ui_squ_2_node_4] -> cal sig21/1(x)
  Constant121/1 -> Mux26/3
  Product7/1 -> Add12/2
  Add14/1 -> Mux26/2
  Abs20/1 -> Mux27/1
  cal d_theta_hat3/3(d_d2ui_hat) -> Integrator12/1
  [ui_sig_4_node_4] -> cal d_theta_hat3/8(ui_sig_4)
  cal sig23/1(z) -> [ui_sig_6_node_4]
  Constant141/1 -> Add12/1
  [ui_sig_1_node_4] -> cal d_theta_hat3/5(ui_sig_1)
  Mux26/1 -> Interpreted MATLAB Function25/1
  Mux27/1 -> Interpreted MATLAB Function23/1
  Constant114/1 -> Product7/1
  [ui_tilt_node_4] -> cal sig22/2(y)
  Mux28/1 -> Interpreted MATLAB Function26/1
  Constant155/1 -> cal d_theta_hat4/4(chi_t)
  [ui_squ_2_node_5] -> cal sig27/1(x)
  Interpreted MATLAB Function33/1 -> trans to column33/1(x)
  choose ui agent 5/1(y) -> Add17/2
  Constant151/1 -> Mux34/2
  [ui_sig_6_node_5] -> cal d_theta_hat4/10(ui_sig_6)
  [ui_squ_4_node_5] -> cal sig24/1(x)
  Integrator15/1 -> Display36/1, Demux16/1, [d2_ui_hat_node_5]
  Constant154/1 -> Product8/1
  [ui_hat_node_5] -> Add17/1
  trans to column31/1(y) -> [ui_squ_1_node_5]
  Constant157/1 -> Mux33/3
  Integrator14/1 -> Display35/1, Demux11/1, [d_ui_hat_node_5]
  Constant145/1 -> cal d_theta_hat4/1(c1)
  Abs28/1 -> Mux34/1
  trans to column34/1(y) -> [ui_squ_6_node_5]
  [ui_tilt_node_5] -> cal sig24/2(y)
  Integrator13/1 -> Display34/1, [ui_hat_node_5]
  cal sig26/1(z) -> [ui_sig_1_node_5]
  Constant148/1 -> cal d_theta_hat4/3(c3)
  Mux35/1 -> Interpreted MATLAB Function33/1
  [ui_tilt_node_5] -> Abs29/1
  [ui_sig_5_node_5] -> cal d_theta_hat4/9(ui_sig_5)
  cal sig27/1(z) -> [ui_sig_2_node_5]
  Constant153/1 -> Add19/1
  Constant150/1 -> Mux34/3
  Abs24/1 -> Mux30/1
  Mux30/1 -> Interpreted MATLAB Function34/1
  Interpreted MATLAB Function29/1 -> trans to column31/1(x)
  trans to column30/1(y) -> [ui_squ_2_node_5]
  Abs27/1 -> Mux32/1
  Add16/1 -> Mux30/2
  Add19/1 -> Mux35/2
  Constant158/1 -> Mux30/3
  [ui_tilt_node_5] -> Abs24/1
  Abs29/1 -> Mux35/1
  Constant146/1 -> cal d_theta_hat4/2(c2)
  Interpreted MATLAB Function30/1 -> trans to column29/1(x)
  [ui_squ_5_node_5] -> cal sig25/1(x)
  trans to column29/1(y) -> [ui_squ_5_node_5]
  Product8/1 -> Add19/2
  Constant143/1 -> Mux31/3
  Add17/1 -> Demux6/1, [ui_tilt_node_5]
  cal d_theta_hat4/2(d_dui_hat) -> Integrator14/1
  Abs25/1 -> Mux31/1
  cal d_theta_hat4/1(d_ui_hat) -> Integrator13/1
  Interpreted MATLAB Function34/1 -> trans to column34/1(x)
  Interpreted MATLAB Function32/1 -> trans to column32/1(x)
  [ui_squ_6_node_5] -> cal sig29/1(x)
  Constant173/1 -> Product8/2
  cal sig24/1(z) -> [ui_sig_4_node_5]
  Constant156/1 -> Mux33/2
  [ui_tilt_node_5] -> cal sig26/2(y)
  trans to column33/1(y) -> [ui_squ_4_node_5]
  Constant147/1 -> Add18/1
  cal sig25/1(z) -> [ui_sig_5_node_5]
  [ui_sig_3_node_5] -> cal d_theta_hat4/7(ui_sig_3)
  Mux31/1 -> Interpreted MATLAB Function30/1
  [ui_tilt_node_5] -> Abs25/1
  [ui_tilt_node_5] -> Abs28/1
  Constant144/1 -> Mux31/2
  [ui_tilt_node_5] -> cal sig25/2(y)
  [ui_tilt_node_5] -> Abs27/1
  Interpreted MATLAB Function31/1 -> trans to column30/1(x)
  [d_ui_hat_node_5] -> cal d_theta_hat4/11(dui_hat)
  Constant172/1 -> Add18/2
  [ui_tilt_node_5] -> Abs26/1
  trans to column32/1(y) -> [ui_squ_3_node_5]
  [ui_squ_3_node_5] -> cal sig28/1(x)
  Constant152/1 -> Mux35/3
  [ui_sig_2_node_5] -> cal d_theta_hat4/6(ui_sig_2)
  [ui_vec] -> choose ui agent 5/1(x)
  [ui_squ_1_node_5] -> cal sig26/1(x)
  [ui_tilt_node_5] -> cal sig28/2(y)
  cal sig28/1(z) -> [ui_sig_3_node_5]
  Constant142/1 -> Product9/1
  Constant159/1 -> Add16/1
  [ui_sig_1_node_5] -> cal d_theta_hat4/5(ui_sig_1)
  Mux32/1 -> Interpreted MATLAB Function31/1
  Mux33/1 -> Interpreted MATLAB Function29/1
  Mux34/1 -> Interpreted MATLAB Function32/1
  Product9/1 -> Add16/2
  cal sig29/1(z) -> [ui_sig_6_node_5]
  Add18/1 -> Mux32/2
  Constant174/1 -> Product9/2
  Constant149/1 -> Mux32/3
  [d2_ui_hat_node_5] -> cal d_theta_hat4/12(d2ui_hat)
  Abs26/1 -> Mux33/1
  cal d_theta_hat4/3(d_d2ui_hat) -> Integrator15/1
  [ui_tilt_node_5] -> cal sig27/2(y)
  [ui_tilt_node_5] -> cal sig29/2(y)
  [ui_sig_4_node_5] -> cal d_theta_hat4/8(ui_sig_4)
  combine duihat d2uihat/2(d2uihat_vec) -> [d2uihat_vec]
  combine duihat d2uihat/1(duihat_vec) -> [duihat_vec]
  [d_ui_hat_node_1] -> combine duihat d2uihat/1(d_ui_hat_node_1)
  [d_ui_hat_node_2] -> combine duihat d2uihat/2(d_ui_hat_node_2)
  [d_ui_hat_node_3] -> combine duihat d2uihat/3(d_ui_hat_node_3)
  [d_ui_hat_node_4] -> combine duihat d2uihat/4(d_ui_hat_node_4)
  [d_ui_hat_node_5] -> combine duihat d2uihat/5(d_ui_hat_node_5)
  [d2_ui_hat_node_1] -> combine duihat d2uihat/6(d2_ui_hat_node_1)
  [d2_ui_hat_node_2] -> combine duihat d2uihat/7(d2_ui_hat_node_2)
  [d2_ui_hat_node_3] -> combine duihat d2uihat/8(d2_ui_hat_node_3)
  [d2_ui_hat_node_4] -> combine duihat d2uihat/9(d2_ui_hat_node_4)
  [d2_ui_hat_node_5] -> combine duihat d2uihat/10(d2_ui_hat_node_5)
  [ui_vec] -> cal wci dwci agent 1/1(ui_vec)
  [duihat_vec] -> cal wci dwci agent 1/2(duihat_vec)
  [d2uihat_vec] -> cal wci dwci agent 1/3(d2uihat_vec)
  [Rci_vec] -> cal wci dwci agent 1/4(Rci_mat)
  cal wci dwci agent 1/2(dwci) -> Display45/1, Demux18/1, [dwci_node_1]
  [ui_vec] -> cal wci dwci agent 2/1(ui_vec)
  cal wci dwci agent 2/2(dwci) -> Display47/1, Demux20/1, [dwci_node_2]
  cal wci dwci agent 2/1(wci) -> Demux19/1, Display46/1, [wci_node_2]
  [d2uihat_vec] -> cal wci dwci agent 2/3(d2uihat_vec)
  [Rci_vec] -> cal wci dwci agent 2/4(Rci_mat)
  [duihat_vec] -> cal wci dwci agent 2/2(duihat_vec)
  [Rci_vec] -> cal wci dwci agent 3/4(Rci_mat)
  cal wci dwci agent 3/1(wci) -> Display48/1, Demux42/1, [wci_node_3]
  [ui_vec] -> cal wci dwci agent 3/1(ui_vec)
  [duihat_vec] -> cal wci dwci agent 3/2(duihat_vec)
  [d2uihat_vec] -> cal wci dwci agent 3/3(d2uihat_vec)
  [Rci_vec] -> cal wci dwci agent 4/4(Rci_mat)
  [ui_vec] -> cal wci dwci agent 4/1(ui_vec)
  [duihat_vec] -> cal wci dwci agent 4/2(duihat_vec)
  cal wci dwci agent 4/1(wci) -> Display50/1, Demux44/1, [wci_node_4]
  cal wci dwci agent 4/2(dwci) -> Display51/1, Demux45/1, [dwci_node_4]
  [d2uihat_vec] -> cal wci dwci agent 4/3(d2uihat_vec)
  cal wci dwci agent 5/1(wci) -> Display52/1, Demux46/1, [wci_node_5]
  [d2uihat_vec] -> cal wci dwci agent 5/3(d2uihat_vec)
  [Rci_vec] -> cal wci dwci agent 5/4(Rci_mat)
  [duihat_vec] -> cal wci dwci agent 5/2(duihat_vec)
  cal wci dwci agent 5/2(dwci) -> Display53/1, Demux47/1, [dwci_node_5]
  [ui_vec] -> cal wci dwci agent 5/1(ui_vec)
  [wci_node_1] -> combine wci dwci/1(wci_node_1)
  [wci_node_2] -> combine wci dwci/2(wci_node_2)
  [wci_node_3] -> combine wci dwci/3(wci_node_3)
  [wci_node_4] -> combine wci dwci/4(wci_node_4)
  [wci_node_5] -> combine wci dwci/5(wci_node_5)
  [dwci_node_1] -> combine wci dwci/6(dwci_node_1)
  [dwci_node_2] -> combine wci dwci/7(dwci_node_2)
  [dwci_node_3] -> combine wci dwci/8(dwci_node_3)
  [dwci_node_4] -> combine wci dwci/9(dwci_node_4)
  [dwci_node_5] -> combine wci dwci/10(dwci_node_5)
  [Qci_vec] -> To Workspace11/1
  [Qi_vec] -> To Workspace20/1
  [Qei_vec] -> To Workspace19/1
  [weitilt_vec] -> To Workspace16/1
  [wei_vec] -> To Workspace13/1
  [wci_vec] -> To Workspace/1
  [wi_vec] -> To Workspace2/1
  Demux2/2 -> ui_tilt_node_1/2
  Demux2/3 -> ui_tilt_node_1/3
  Demux2/1 -> ui_tilt_node_1/1
  Demux3/3 -> ui_tilt_node_2/3
  Demux3/1 -> ui_tilt_node_2/1
  Demux3/2 -> ui_tilt_node_2/2
  Demux4/3 -> ui_tilt_node_3/3
  Demux4/1 -> ui_tilt_node_3/1
  Demux4/2 -> ui_tilt_node_3/2
  Demux5/3 -> ui_tilt_node_4/3
  Demux5/1 -> ui_tilt_node_4/1
  Demux5/2 -> ui_tilt_node_4/2
  Demux6/3 -> ui_tilt_node_5/3
  Demux6/1 -> ui_tilt_node_5/1
  Demux6/2 -> ui_tilt_node_5/2
  Demux7/3 -> d_ui_hat_node_3/3
  Demux7/1 -> d_ui_hat_node_3/1
  Demux7/2 -> d_ui_hat_node_3/2
  Demux8/2 -> d_ui_hat_node_1/2
  Demux8/1 -> d_ui_hat_node_1/1
  Demux8/3 -> d_ui_hat_node_1/3
  Demux9/2 -> d_ui_hat_node_2/2
  Demux9/1 -> d_ui_hat_node_2/1
  Demux9/3 -> d_ui_hat_node_2/3
  Integrator5/1 -> Display26/1, [d_ui_hat_node_2], Demux9/1
  Demux10/2 -> d_ui_hat_node_4/2
  Demux10/1 -> d_ui_hat_node_4/1
  Demux10/3 -> d_ui_hat_node_4/3
  Demux11/2 -> d_ui_hat_node_5/2
  Demux11/1 -> d_ui_hat_node_5/1
  Demux11/3 -> d_ui_hat_node_5/3
  Demux12/2 -> d2_ui_hat_node_1/2
  Demux12/1 -> d2_ui_hat_node_1/1
  Demux12/3 -> d2_ui_hat_node_1/3
  Demux13/3 -> d2_ui_hat_node_2/3
  Demux13/2 -> d2_ui_hat_node_2/2
  Demux13/1 -> d2_ui_hat_node_2/1
  Demux14/3 -> d2_ui_hat_node_3/3
  Demux14/2 -> d2_ui_hat_node_3/2
  Demux14/1 -> d2_ui_hat_node_3/1
  Demux15/3 -> d2_ui_hat_node_4/3
  Demux15/2 -> d2_ui_hat_node_4/2
  Demux15/1 -> d2_ui_hat_node_4/1
  Demux16/3 -> d2_ui_hat_node_5/3
  Demux16/2 -> d2_ui_hat_node_5/2
  Demux16/1 -> d2_ui_hat_node_5/1
  Demux17/3 -> wci_node_1/3
  Demux17/1 -> wci_node_1/1
  Demux17/2 -> wci_node_1/2
  Demux18/1 -> dwci_node_1/1
  Demux18/2 -> dwci_node_1/2
  Demux18/3 -> dwci_node_1/3
  Demux19/2 -> wci_node_2/2
  Demux19/1 -> wci_node_2/1
  Demux19/3 -> wci_node_2/3
  Demux20/2 -> dwci_node_2/2
  Demux20/1 -> dwci_node_2/1
  Demux20/3 -> dwci_node_2/3
  Demux42/3 -> wci_node_3/3
  Demux42/2 -> wci_node_3/2
  Demux42/1 -> wci_node_3/1
  Demux43/3 -> dwci_node_3/3
  Demux43/2 -> dwci_node_3/2
  Demux43/1 -> dwci_node_3/1
  Demux44/3 -> wci_node_4/3
  Demux44/2 -> wci_node_4/2
  Demux44/1 -> wci_node_4/1
  Demux45/3 -> dwci_node_4/3
  Demux45/1 -> dwci_node_4/1
  Demux45/2 -> dwci_node_4/2
  Demux46/3 -> wci_node_5/3
  Demux46/1 -> wci_node_5/1
  Demux46/2 -> wci_node_5/2
  Demux47/3 -> dwci_node_5/3
  Demux47/1 -> dwci_node_5/1
  Demux47/2 -> dwci_node_5/2
  cal wci dwci agent 1/1(wci) -> Display44/1, Demux17/1, [wci_node_1]
  cal wci dwci agent 3/2(dwci) -> [dwci_node_3], Display49/1, Demux43/1
  combine wci dwci/1(wci_vec) -> Memory14/1
  combine wci dwci/2(dwci_vec) -> Memory15/1
  [ui_hat_node_4] -> Demux53/1
  Demux48/3 -> Mux43/2
  Demux56/2 -> Mux54/2
  Demux54/3 -> Mux49/2
  Mux50/1 -> Scope14/1
  Demux48/2 -> Mux42/2
  Demux49/1 -> Mux48/1
  Mux54/1 -> Scope15/2
  Demux50/1 -> Mux48/2
  Demux55/2 -> Mux54/1
  Mux49/1 -> Scope14/3
  Demux51/2 -> Mux47/1
  [ui_5] -> Demux56/1
  [ui_hat_node_5] -> Demux55/1
  Mux53/1 -> Scope15/1
  [ui_4] -> Demux54/1
  Demux52/2 -> Mux47/2
  Mux52/1 -> Scope15/3
  Demux53/1 -> Mux50/1
  Demux55/1 -> Mux53/1
  Demux54/1 -> Mux50/2
  Demux54/2 -> Mux51/2
  Mux45/1 -> Scope13/3
  [ui_3] -> Demux52/1
  Demux52/3 -> Mux45/2
  Demux51/3 -> Mux45/1
  [ui_1] -> Demux48/1
  Demux55/3 -> Mux52/1
  Demux50/2 -> Mux55/2
  Mux46/1 -> Scope13/1
  Mux42/1 -> Scope2/2
  Demux52/1 -> Mux46/2
  Demux56/1 -> Mux53/2
  [ui_hat_node_3] -> Demux51/1
  [ui_hat_node_2] -> Demux49/1
  Demux/2 -> Mux42/1
  Mux48/1 -> Scope1/1
  Demux49/3 -> Mux44/1
  Demux49/2 -> Mux55/1
  Mux44/1 -> Scope1/3
  Mux47/1 -> Scope13/2
  Demux/3 -> Mux43/1
  [ui_2] -> Demux50/1
  Mux43/1 -> Scope2/3
  Demux53/3 -> Mux49/1
  Mux51/1 -> Scope14/2
  Mux55/1 -> Scope1/2
  Demux56/3 -> Mux52/2
  Mux41/1 -> Scope2/1
  Demux53/2 -> Mux51/1
  Demux/1 -> Mux41/1
  [ui_hat_node_1] -> Demux/1
  Demux50/3 -> Mux44/2
  Demux51/1 -> Mux46/1
  Demux48/1 -> Mux41/2
  Constant1/1 -> cal d_sigma_w agent 1/1(h3w)
  Constant2/1 -> cal d_sigma_w agent 1/2(Ji)
  [wi_vec] -> cal d_sigma_w agent 1/3(wi_vec)
  [taui_vec] -> cal d_sigma_w agent 1/4(taui_vec)
  [sigma_bar_w_vec] -> cal d_sigma_w agent 1/5(sigma_w_bar_vec)
  Constant4/1 -> cal d_sigma_w agent 2/2(Ji)
  Constant3/1 -> cal d_sigma_w agent 2/1(h3w)
  [wi_vec] -> cal d_sigma_w agent 2/3(wi_vec)
  [sigma_bar_w_vec] -> cal d_sigma_w agent 2/5(sigma_w_bar_vec)
  [taui_vec] -> cal d_sigma_w agent 2/4(taui_vec)
  cal d_sigma_w agent 2/1(d_sigma_w_2) -> Integrator17/1
  [sigma_bar_w_vec] -> cal d_sigma_w agent 3/5(sigma_w_bar_vec)
  cal d_sigma_w agent 3/1(d_sigma_w_3) -> Integrator18/1
  Constant6/1 -> cal d_sigma_w agent 3/2(Ji)
  Constant5/1 -> cal d_sigma_w agent 3/1(h3w)
  [taui_vec] -> cal d_sigma_w agent 3/4(taui_vec)
  [wi_vec] -> cal d_sigma_w agent 3/3(wi_vec)
  Constant7/1 -> cal d_sigma_w agent 4/1(h3w)
  cal d_sigma_w agent 4/1(d_sigma_w_4) -> Integrator19/1
  Constant8/1 -> cal d_sigma_w agent 4/2(Ji)
  [wi_vec] -> cal d_sigma_w agent 4/3(wi_vec)
  [taui_vec] -> cal d_sigma_w agent 4/4(taui_vec)
  [sigma_bar_w_vec] -> cal d_sigma_w agent 4/5(sigma_w_bar_vec)
  [wi_vec] -> cal d_sigma_w agent 5/3(wi_vec)
  [sigma_bar_w_vec] -> cal d_sigma_w agent 5/5(sigma_w_bar_vec)
  Constant10/1 -> cal d_sigma_w agent 5/2(Ji)
  cal d_sigma_w agent 5/1(d_sigma_w_5) -> Integrator20/1
  Constant9/1 -> cal d_sigma_w agent 5/1(h3w)
  [taui_vec] -> cal d_sigma_w agent 5/4(taui_vec)
  cal d_sigma_w agent 1/1(d_sigma_w_1) -> Integrator16/1
  Integrator16/1 -> [sigma_w_1]
  Integrator17/1 -> [sigma_w_2]
  Integrator18/1 -> [sigma_w_3]
  Integrator19/1 -> [sigma_w_4]
  Integrator20/1 -> [sigma_w_5]
  [sigma_w_1] -> combine sigma_w/1(sigma_w_1)
  [sigma_w_2] -> combine sigma_w/2(sigma_w_2)
  [sigma_w_3] -> combine sigma_w/3(sigma_w_3)
  [sigma_w_4] -> combine sigma_w/4(sigma_w_4)
  [sigma_w_5] -> combine sigma_w/5(sigma_w_5)
  combine sigma_w/1(sigma_w_vec) -> [sigma_w_vec]
  [wi_vec] -> cal sigma_w_bar/1(wi_vec)
  [sigma_w_vec] -> cal sigma_w_bar/2(sigma_w_vec)
  cal sigma_w_bar/1(sigma_bar_w_vec) -> [sigma_bar_w_vec]
  Demux24/1 -> d_sigma_bar_w_est_1/1
  cal differentiator d_sigma_bar_w_hat agent 1/3(Out3) -> Demux23/1, [d2_sigma_bar_w_est_1], Display37/1
  Demux24/2 -> d_sigma_bar_w_est_1/2
  Demux23/3 -> d2_sigma_bar_w_est_1/3
  cal differentiator d_sigma_bar_w_hat agent 1/1(Out1) -> Display1/1, [sigma_bar_w_est_1]
  Demux23/2 -> d2_sigma_bar_w_est_1/2
  cal differentiator d_sigma_bar_w_hat agent 1/2(Out2) -> Demux24/1, [d_sigma_bar_w_est_1], Display2/1
  [sigma_bar_w_vec] -> cal differentiator d_sigma_bar_w_hat agent 1/1(x)
  Demux24/3 -> d_sigma_bar_w_est_1/3
  Demux23/1 -> d2_sigma_bar_w_est_1/1
  Demux25/3 -> d2_sigma_bar_w_est_2/3
  Demux26/2 -> d_sigma_bar_w_est_2/2
  cal differentiator d_sigma_bar_w_hat agent 2/3(Out3) -> Demux25/1, [d2_sigma_bar_w_est_2], Display5/1
  Demux26/1 -> d_sigma_bar_w_est_2/1
  Demux25/2 -> d2_sigma_bar_w_est_2/2
  Demux25/1 -> d2_sigma_bar_w_est_2/1
  Demux26/3 -> d_sigma_bar_w_est_2/3
  cal differentiator d_sigma_bar_w_hat agent 2/1(Out1) -> Display3/1, [sigma_bar_w_est_2]
  [sigma_bar_w_vec] -> cal differentiator d_sigma_bar_w_hat agent 2/1(x)
  cal differentiator d_sigma_bar_w_hat agent 2/2(Out2) -> Demux26/1, [d_sigma_bar_w_est_2], Display4/1
  cal differentiator d_sigma_bar_w_hat agent 3/2(Out2) -> Demux28/1, [d_sigma_bar_w_est_3], Display7/1
  [sigma_bar_w_vec] -> cal differentiator d_sigma_bar_w_hat agent 3/1(x)
  cal differentiator d_sigma_bar_w_hat agent 3/1(Out1) -> Display6/1, [sigma_bar_w_est_3]
  Demux27/2 -> d2_sigma_bar_w_est_3/2
  Demux27/1 -> d2_sigma_bar_w_est_3/1
  Demux28/3 -> d_sigma_bar_w_est_3/3
  cal differentiator d_sigma_bar_w_hat agent 3/3(Out3) -> Demux27/1, [d2_sigma_bar_w_est_3], Display8/1
  Demux27/3 -> d2_sigma_bar_w_est_3/3
  Demux28/2 -> d_sigma_bar_w_est_3/2
  Demux28/1 -> d_sigma_bar_w_est_3/1
  cal differentiator d_sigma_bar_w_hat agent 4/3(Out3) -> Demux29/1, [d2_sigma_bar_w_est_4], Display11/1
  Demux29/3 -> d2_sigma_bar_w_est_4/3
  Demux30/2 -> d_sigma_bar_w_est_4/2
  [sigma_bar_w_vec] -> cal differentiator d_sigma_bar_w_hat agent 4/1(x)
  Demux30/1 -> d_sigma_bar_w_est_4/1
  Demux29/2 -> d2_sigma_bar_w_est_4/2
  Demux29/1 -> d2_sigma_bar_w_est_4/1
  Demux30/3 -> d_sigma_bar_w_est_4/3
  cal differentiator d_sigma_bar_w_hat agent 4/2(Out2) -> Demux30/1, [d_sigma_bar_w_est_4], Display10/1
  cal differentiator d_sigma_bar_w_hat agent 4/1(Out1) -> Display9/1, [sigma_bar_w_est_4]
  Demux32/3 -> d_sigma_bar_w_est_5/3
  Demux31/2 -> d2_sigma_bar_w_est_5/2
  Demux31/1 -> d2_sigma_bar_w_est_5/1
  Demux32/1 -> d_sigma_bar_w_est_5/1
  Demux32/2 -> d_sigma_bar_w_est_5/2
  [sigma_bar_w_vec] -> cal differentiator d_sigma_bar_w_hat agent 5/1(x)
  cal differentiator d_sigma_bar_w_hat agent 5/1(Out1) -> Display14/1, [sigma_bar_w_est_5]
  cal differentiator d_sigma_bar_w_hat agent 5/2(Out2) -> Demux32/1, [d_sigma_bar_w_est_5], Display12/1
  Demux31/3 -> d2_sigma_bar_w_est_5/3
  cal differentiator d_sigma_bar_w_hat agent 5/3(Out3) -> Demux31/1, [d2_sigma_bar_w_est_5], Display13/1
  [d_sigma_bar_w_est_3] -> combine d_sigma_bar_v_est/3(d_sigma_bar_w_est_3)
  [d_sigma_bar_w_est_5] -> combine d_sigma_bar_v_est/5(d_sigma_bar_w_est_5)
  [d_sigma_bar_w_est_4] -> combine d_sigma_bar_v_est/4(d_sigma_bar_w_est_4)
  [d_sigma_bar_w_est_1] -> combine d_sigma_bar_v_est/1(d_sigma_bar_w_est_1)
  [d_sigma_bar_w_est_2] -> combine d_sigma_bar_v_est/2(d_sigma_bar_w_est_2)
  combine d_sigma_bar_v_est/1(d_sigma_bar_w_vec) -> [d_sigma_bar_w_vec]
  choose ksi_est_err 30/1(y) -> cal abs 30/1(x)
  Mux39/1 -> Interpreted MATLAB Function38/1
  Mux37/1 -> Interpreted MATLAB Function36/1
  [sigma_bar_w_tilt_vec] -> cal theta_sigma_bar_w_tilt agent 2/4(sigma_bar_w_tilt_vec)
  Constant16/1 -> Mux3/2
  Constant30/1 -> Mux40/3
  Constant17/1 -> Mux3/3
  cal abs 29/1(y) -> Mux40/1
  Constant31/1 -> Mux39/2
  [sigma_bar_w_tilt_vec] -> choose ksi_est_err 24/1(x)
  Interpreted MATLAB Function38/1 -> trans to column39/1(x)
  trans to column4/1(y) -> [sigma_bar_w_tilt_squ_1_2], Display18/1
  combine theta_sigma_bar_w_tilt/2(theta_sigma_bar_w_tilt_2_vec) -> [theta_sigma_bar_w_tilt_2_vec]
  Constant33/1 -> Mux2/3
  Mux4/1 -> Interpreted MATLAB Function4/1
  [sigma_bar_w_tilt_vec] -> choose ksi_est_err 30/1(x)
  Constant34/1 -> Mux1/2
  [sigma_bar_w_tilt_vec] -> choose ksi_est_err 25/1(x)
  [sigma_bar_w_tilt_squ_2_5] -> cal theta_sigma_bar_w_tilt agent 5/3(sigma_bar_w_tilt_squ_2_5)
  cal abs 21/1(y) -> Mux2/1
  [sigma_bar_w_tilt_vec] -> choose ksi_est_err 23/1(x)
  Interpreted MATLAB Function35/1 -> trans to column36/1(x)
  choose ksi_est_err 24/1(y) -> cal abs 24/1(x)
  choose ksi_est_err 29/1(y) -> cal abs 29/1(x)
  [sigma_bar_w_tilt_vec] -> choose ksi_est_err 21/1(x)
  trans to column36/1(y) -> [sigma_bar_w_tilt_squ_1_3], Display20/1
  trans to column38/1(y) -> [sigma_bar_w_tilt_squ_1_4], Display39/1
  Mux1/1 -> Interpreted MATLAB Function1/1
  [sigma_bar_w_tilt_squ_2_3] -> cal theta_sigma_bar_w_tilt agent 3/3(sigma_bar_w_tilt_squ_2_3)
  cal abs 28/1(y) -> Mux37/1
  [theta_sigma_bar_w_tilt_1_2] -> combine theta_sigma_bar_w_tilt/2(theta_sigma_bar_w_tilt_1_2)
  [sigma_bar_w_tilt_squ_2_1] -> cal theta_sigma_bar_w_tilt agent 1/3(sigma_bar_w_tilt_squ_2_1)
  cal theta_sigma_bar_w_tilt agent 1/2(theta_sigma_bar_w_tilt_2_1) -> [theta_sigma_bar_w_tilt_2_1]
  Constant13/1 -> Mux4/2
  Constant28/1 -> Mux40/2
  trans to column1/1(y) -> [sigma_bar_w_tilt_squ_2_1], Display15/1
  [theta_sigma_bar_w_tilt_2_3] -> combine theta_sigma_bar_w_tilt/8(theta_sigma_bar_w_tilt_2_3)
  [theta_sigma_bar_w_tilt_1_4] -> combine theta_sigma_bar_w_tilt/4(theta_sigma_bar_w_tilt_1_4)
  [theta_sigma_bar_w_tilt_2_4] -> combine theta_sigma_bar_w_tilt/9(theta_sigma_bar_w_tilt_2_4)
  [theta_sigma_bar_w_tilt_1_3] -> combine theta_sigma_bar_w_tilt/3(theta_sigma_bar_w_tilt_1_3)
  [theta_sigma_bar_w_tilt_2_2] -> combine theta_sigma_bar_w_tilt/7(theta_sigma_bar_w_tilt_2_2)
  [theta_sigma_bar_w_tilt_1_1] -> combine theta_sigma_bar_w_tilt/1(theta_sigma_bar_w_tilt_1_1)
  [theta_sigma_bar_w_tilt_2_5] -> combine theta_sigma_bar_w_tilt/10(theta_sigma_bar_w_tilt_2_5)
  Interpreted MATLAB Function39/1 -> trans to column40/1(x)
  combine theta_sigma_bar_w_tilt/1(theta_sigma_bar_w_tilt_1_vec) -> [theta_sigma_bar_w_tilt_1_vec]
  cal abs 30/1(y) -> Mux39/1
  [sigma_bar_w_tilt_vec] -> choose ksi_est_err 29/1(x)
  [sigma_bar_w_tilt_vec] -> choose ksi_est_err 27/1(x)
  Constant32/1 -> Mux39/3
  trans to column39/1(y) -> [sigma_bar_w_tilt_squ_2_5], Display40/1
  [theta_sigma_bar_w_tilt_2_1] -> combine theta_sigma_bar_w_tilt/6(theta_sigma_bar_w_tilt_2_1)
  cal theta_sigma_bar_w_tilt agent 5/2(theta_sigma_bar_w_tilt_2_5) -> [theta_sigma_bar_w_tilt_2_5]
  Constant29/1 -> cal theta_sigma_bar_w_tilt agent 5/1(alfa_theta_obs_w)
  Mux40/1 -> Interpreted MATLAB Function39/1
  cal theta_sigma_bar_w_tilt agent 5/1(theta_sigma_bar_w_tilt_1_5) -> [theta_sigma_bar_w_tilt_1_5]
  cal theta_sigma_bar_w_tilt agent 4/2(theta_sigma_bar_w_tilt_2_4) -> [theta_sigma_bar_w_tilt_2_4]
  cal theta_sigma_bar_w_tilt agent 4/1(theta_sigma_bar_w_tilt_1_4) -> [theta_sigma_bar_w_tilt_1_4]
  [sigma_bar_w_tilt_squ_2_4] -> cal theta_sigma_bar_w_tilt agent 4/3(sigma_bar_w_tilt_squ_2_4)
  Interpreted MATLAB Function36/1 -> trans to column37/1(x)
  [sigma_bar_w_tilt_vec] -> choose ksi_est_err 28/1(x)
  Interpreted MATLAB Function5/1 -> trans to column35/1(x)
  cal abs 27/1(y) -> Mux38/1
  cal theta_sigma_bar_w_tilt agent 1/1(theta_sigma_bar_w_tilt_1_1) -> [theta_sigma_bar_w_tilt_1_1]
  [sigma_bar_w_tilt_vec] -> cal theta_sigma_bar_w_tilt agent 4/4(sigma_bar_w_tilt_vec)
  [sigma_bar_w_tilt_squ_1_4] -> cal theta_sigma_bar_w_tilt agent 4/2(sigma_bar_w_tilt_squ_1_4)
  Constant27/1 -> Mux37/3
  [sigma_bar_w_tilt_vec] -> cal theta_sigma_bar_w_tilt agent 3/4(sigma_bar_w_tilt_vec)
  [sigma_bar_w_tilt_vec] -> choose ksi_est_err 26/1(x)
  cal theta_sigma_bar_w_tilt agent 2/2(theta_sigma_bar_w_tilt_2_2) -> [theta_sigma_bar_w_tilt_2_2]
  Constant22/1 -> Mux5/3
  Constant19/1 -> cal theta_sigma_bar_w_tilt agent 3/1(alfa_theta_obs_w)
  cal theta_sigma_bar_w_tilt agent 3/1(theta_sigma_bar_w_tilt_1_3) -> [theta_sigma_bar_w_tilt_1_3]
  Constant18/1 -> Mux36/2
  choose ksi_est_err 26/1(y) -> cal abs 26/1(x)
  cal abs 24/1(y) -> Mux3/1
  cal abs 23/1(y) -> Mux4/1
  choose ksi_est_err 25/1(y) -> cal abs 25/1(x)
  choose ksi_est_err 23/1(y) -> cal abs 23/1(x)
  Constant15/1 -> Mux4/3
  Interpreted MATLAB Function3/1 -> trans to column3/1(x)
  [sigma_bar_w_tilt_squ_2_2] -> cal theta_sigma_bar_w_tilt agent 2/3(sigma_bar_w_tilt_squ_2_2)
  trans to column37/1(y) -> [sigma_bar_w_tilt_squ_2_4], Display21/1
  Constant21/1 -> Mux5/2
  trans to column3/1(y) -> [sigma_bar_w_tilt_squ_2_2], Display17/1
  cal theta_sigma_bar_w_tilt agent 2/1(theta_sigma_bar_w_tilt_1_2) -> [theta_sigma_bar_w_tilt_1_2]
  Constant25/1 -> Mux38/3
  Interpreted MATLAB Function4/1 -> trans to column4/1(x)
  choose ksi_est_err 22/1(y) -> cal abs 22/1(x)
  Mux2/1 -> Interpreted MATLAB Function2/1
  choose ksi_est_err 21/1(y) -> cal abs 21/1(x)
  [theta_sigma_bar_w_tilt_1_5] -> combine theta_sigma_bar_w_tilt/5(theta_sigma_bar_w_tilt_1_5)
  Constant23/1 -> Mux38/2
  Interpreted MATLAB Function1/1 -> trans to column1/1(x)
  Constant20/1 -> Mux36/3
  choose ksi_est_err 27/1(y) -> cal abs 27/1(x)
  Constant12/1 -> cal theta_sigma_bar_w_tilt agent 1/1(alfa_theta_obs_w)
  Mux38/1 -> Interpreted MATLAB Function37/1
  [sigma_bar_w_tilt_vec] -> cal theta_sigma_bar_w_tilt agent 1/4(sigma_bar_w_tilt_vec)
  Constant14/1 -> cal theta_sigma_bar_w_tilt agent 2/1(alfa_theta_obs_w)
  Constant35/1 -> Mux1/3
  [sigma_bar_w_tilt_vec] -> choose ksi_est_err 22/1(x)
  [sigma_bar_w_tilt_squ_1_1] -> cal theta_sigma_bar_w_tilt agent 1/2(sigma_bar_w_tilt_squ_1_1)
  Constant11/1 -> Mux2/2
  [sigma_bar_w_tilt_squ_1_3] -> cal theta_sigma_bar_w_tilt agent 3/2(sigma_bar_w_tilt_squ_1_3)
  Mux36/1 -> Interpreted MATLAB Function35/1
  trans to column40/1(y) -> [sigma_bar_w_tilt_squ_1_5], Display41/1
  Constant24/1 -> cal theta_sigma_bar_w_tilt agent 4/1(alfa_theta_obs_w)
  Mux3/1 -> Interpreted MATLAB Function3/1
  cal abs 25/1(y) -> Mux36/1
  cal theta_sigma_bar_w_tilt agent 3/2(theta_sigma_bar_w_tilt_2_3) -> [theta_sigma_bar_w_tilt_2_3]
  [sigma_bar_w_tilt_squ_1_5] -> cal theta_sigma_bar_w_tilt agent 5/2(sigma_bar_w_tilt_squ_1_5)
  trans to column2/1(y) -> [sigma_bar_w_tilt_squ_1_1], Display16/1
  trans to column35/1(y) -> [sigma_bar_w_tilt_squ_2_3], Display19/1
  Constant26/1 -> Mux37/2
  choose ksi_est_err 28/1(y) -> cal abs 28/1(x)
  [sigma_bar_w_tilt_vec] -> cal theta_sigma_bar_w_tilt agent 5/4(sigma_bar_w_tilt_vec)
  [sigma_bar_w_tilt_squ_1_2] -> cal theta_sigma_bar_w_tilt agent 2/2(sigma_bar_w_tilt_squ_1_2)
  cal abs 22/1(y) -> Mux1/1
  Mux5/1 -> Interpreted MATLAB Function5/1
  Interpreted MATLAB Function2/1 -> trans to column2/1(x)
  Interpreted MATLAB Function37/1 -> trans to column38/1(x)
  cal abs 26/1(y) -> Mux5/1
  cal combine sigma_bar_w_tilt/1(sigma_bar_w_tilt_vec) -> [sigma_bar_w_tilt_vec]
  [sigma_bar_w_hat_4] -> combine sigma_bar_w_hat/4(sigma_bar_w_hat_4)
  cal sigma_bar_w_hat agent 2/1(d_sigma_bar_w_hat_2) -> sigma_bar_w_hat Integrator 2/1
  [d_sigma_bar_w_vec] -> cal sigma_bar_w_hat agent 3/5(d_sigma_bar_w_vec)
  [theta_sigma_bar_w_tilt_2_vec] -> cal sigma_bar_w_hat agent 1/4(theta_sigma_bar_w_tilt_2_vec)
  [sigma_bar_w_hat_2] -> combine sigma_bar_w_hat/2(sigma_bar_w_hat_2)
  [dw_hat_4] -> combine dw_hat/4(dw_hat_4)
  [sigma_bar_w_hat_vec] -> cal combine sigma_bar_w_tilt/2(sigma_bar_w_hat_vec)
  [theta_sigma_bar_w_tilt_2_vec] -> cal sigma_bar_w_hat agent 4/4(theta_sigma_bar_w_tilt_2_vec)
  sigma_bar_w_hat Integrator 5/1 -> [sigma_bar_w_hat_5]
  combine sigma_bar_w_hat/1(sigma_bar_w_hat_vec) -> [sigma_bar_w_hat_vec]
  [d_sigma_bar_w_vec] -> cal dw_hat agent 1/3(d_sigma_bar_w_vec)
  [d_sigma_bar_w_vec] -> cal sigma_bar_w_hat agent 5/5(d_sigma_bar_w_vec)
  [theta_sigma_bar_w_tilt_2_vec] -> cal sigma_bar_w_hat agent 5/4(theta_sigma_bar_w_tilt_2_vec)
  Constant45/1 -> cal sigma_bar_w_hat agent 5/2(h2w)
  combine dw_hat/1(dw_hat_vec) -> [dw_hat_vec]
  Constant46/1 -> cal dw_hat agent 1/1(h3w)
  sigma_bar_w_hat Integrator 2/1 -> [sigma_bar_w_hat_2]
  [theta_sigma_bar_w_tilt_1_vec] -> cal sigma_bar_w_hat agent 4/3(theta_sigma_bar_w_tilt_1_vec)
  [sigma_bar_w_hat_5] -> combine sigma_bar_w_hat/5(sigma_bar_w_hat_5)
  Constant44/1 -> cal sigma_bar_w_hat agent 5/1(h1w)
  [theta_sigma_bar_w_tilt_1_vec] -> cal sigma_bar_w_hat agent 5/3(theta_sigma_bar_w_tilt_1_vec)
  cal sigma_bar_w_hat agent 5/1(d_sigma_bar_w_hat_5) -> sigma_bar_w_hat Integrator 5/1
  [sigma_bar_w_hat_1] -> combine sigma_bar_w_hat/1(sigma_bar_w_hat_1)
  [sigma_bar_w_hat_vec] -> cal dw_hat agent 1/4(sigma_bar_w_hat_vec)
  Constant42/1 -> cal sigma_bar_w_hat agent 4/1(h1w)
  sigma_bar_w_hat Integrator 1/1 -> [sigma_bar_w_hat_1]
  [dw_hat_3] -> combine dw_hat/3(dw_hat_3)
  sigma_bar_w_hat Integrator 3/1 -> [sigma_bar_w_hat_3]
  [sigma_bar_w_hat_3] -> combine sigma_bar_w_hat/3(sigma_bar_w_hat_3)
  [sigma_bar_w_vec] -> cal combine sigma_bar_w_tilt/1(sigma_bar_w_vec)
  [d_sigma_bar_w_vec] -> cal sigma_bar_w_hat agent 2/5(d_sigma_bar_w_vec)
  Constant38/1 -> cal sigma_bar_w_hat agent 2/1(h1w)
  [dw_hat_5] -> combine dw_hat/5(dw_hat_5)
  cal dw_hat agent 1/1(dw_hat_1) -> [dw_hat_1]
  cal sigma_bar_w_hat agent 4/1(d_sigma_bar_w_hat_4) -> sigma_bar_w_hat Integrator 4/1
  [theta_sigma_bar_w_tilt_1_vec] -> cal sigma_bar_w_hat agent 3/3(theta_sigma_bar_w_tilt_1_vec)
  [dw_hat_1] -> combine dw_hat/1(dw_hat_1)
  [theta_sigma_bar_w_tilt_1_vec] -> cal sigma_bar_w_hat agent 2/3(theta_sigma_bar_w_tilt_1_vec)
  Constant40/1 -> cal sigma_bar_w_hat agent 3/1(h1w)
  [theta_sigma_bar_w_tilt_2_vec] -> cal sigma_bar_w_hat agent 2/4(theta_sigma_bar_w_tilt_2_vec)
  [theta_sigma_bar_w_tilt_2_vec] -> cal sigma_bar_w_hat agent 3/4(theta_sigma_bar_w_tilt_2_vec)
  Constant39/1 -> cal sigma_bar_w_hat agent 2/2(h2w)
  cal sigma_bar_w_hat agent 3/1(d_sigma_bar_w_hat_3) -> sigma_bar_w_hat Integrator 3/1
  Constant43/1 -> cal sigma_bar_w_hat agent 4/2(h2w)
  Constant36/1 -> cal sigma_bar_w_hat agent 1/1(h1w)
  [theta_sigma_bar_w_tilt_1_vec] -> cal sigma_bar_w_hat agent 1/3(theta_sigma_bar_w_tilt_1_vec)
  cal sigma_bar_w_hat agent 1/1(d_sigma_bar_w_hat_1) -> sigma_bar_w_hat Integrator 1/1
  [dw_hat_2] -> combine dw_hat/2(dw_hat_2)
  [d_sigma_bar_w_vec] -> cal sigma_bar_w_hat agent 1/5(d_sigma_bar_w_vec)
  [d_sigma_bar_w_vec] -> cal sigma_bar_w_hat agent 4/5(d_sigma_bar_w_vec)
  Constant41/1 -> cal sigma_bar_w_hat agent 3/2(h2w)
  sigma_bar_w_hat Integrator 4/1 -> [sigma_bar_w_hat_4]
  Constant37/1 -> cal sigma_bar_w_hat agent 1/2(h2w)
  Constant64/1 -> cal dw_hat agent 1/2(Ji)
  Constant48/1 -> cal dw_hat agent 2/2(Ji)
  [sigma_bar_w_hat_vec] -> cal dw_hat agent 2/4(sigma_bar_w_hat_vec)
  Constant47/1 -> cal dw_hat agent 2/1(h3w)
  [d_sigma_bar_w_vec] -> cal dw_hat agent 2/3(d_sigma_bar_w_vec)
  cal dw_hat agent 2/1(dw_hat_2) -> [dw_hat_2]
  [d_sigma_bar_w_vec] -> cal dw_hat agent 3/3(d_sigma_bar_w_vec)
  Constant49/1 -> cal dw_hat agent 3/1(h3w)
  [sigma_bar_w_hat_vec] -> cal dw_hat agent 3/4(sigma_bar_w_hat_vec)
  cal dw_hat agent 3/1(dw_hat_3) -> [dw_hat_3]
  Constant50/1 -> cal dw_hat agent 3/2(Ji)
  cal dw_hat agent 4/1(dw_hat_4) -> [dw_hat_4]
  [sigma_bar_w_hat_vec] -> cal dw_hat agent 4/4(sigma_bar_w_hat_vec)
  [d_sigma_bar_w_vec] -> cal dw_hat agent 4/3(d_sigma_bar_w_vec)
  Constant66/1 -> cal dw_hat agent 4/2(Ji)
  Constant65/1 -> cal dw_hat agent 4/1(h3w)
  [d_sigma_bar_w_vec] -> cal dw_hat agent 5/3(d_sigma_bar_w_vec)
  Constant67/1 -> cal dw_hat agent 5/1(h3w)
  Constant68/1 -> cal dw_hat agent 5/2(Ji)
  [sigma_bar_w_hat_vec] -> cal dw_hat agent 5/4(sigma_bar_w_hat_vec)
  cal dw_hat agent 5/1(dw_hat_5) -> [dw_hat_5]
  Constant69/1 -> cal taui agent 1/1(kR)
  Constant70/1 -> cal taui agent 1/2(kRtilt)
  Constant71/1 -> cal taui agent 1/3(Ji)
  [V_Phi_Rei_vec] -> cal taui agent 1/4(V_Phi_Rei_vec)
  [V_Phi_Reitilt_vec] -> cal taui agent 1/5(V_Phi_Reitilt_vec)
  [dw_hat_vec] -> cal taui agent 1/6(dw_hat_vec)
  [Rei_vec] -> cal taui agent 1/7(Rei_vec)
  [wci_vec] -> cal taui agent 1/8(wci_vec)
  [dwci_vec] -> cal taui agent 1/9(dwci_vec)
  cal taui agent 1/1(tau_1) -> [tau_1]
  Constant72/1 -> cal taui agent 2/1(kR)
  [Rei_vec] -> cal taui agent 2/7(Rei_vec)
  [dw_hat_vec] -> cal taui agent 2/6(dw_hat_vec)
  Constant129/1 -> cal taui agent 2/3(Ji)
  [V_Phi_Rei_vec] -> cal taui agent 2/4(V_Phi_Rei_vec)
  [wci_vec] -> cal taui agent 2/8(wci_vec)
  cal taui agent 2/1(tau_2) -> [tau_2]
  [V_Phi_Reitilt_vec] -> cal taui agent 2/5(V_Phi_Reitilt_vec)
  Constant73/1 -> cal taui agent 2/2(kRtilt)
  [dwci_vec] -> cal taui agent 2/9(dwci_vec)
  [dwci_vec] -> cal taui agent 3/9(dwci_vec)
  Constant130/1 -> cal taui agent 3/3(Ji)
  Constant132/1 -> cal taui agent 3/2(kRtilt)
  cal taui agent 3/1(tau_3) -> [tau_3]
  [dw_hat_vec] -> cal taui agent 3/6(dw_hat_vec)
  [V_Phi_Rei_vec] -> cal taui agent 3/4(V_Phi_Rei_vec)
  [V_Phi_Reitilt_vec] -> cal taui agent 3/5(V_Phi_Reitilt_vec)
  [Rei_vec] -> cal taui agent 3/7(Rei_vec)
  Constant131/1 -> cal taui agent 3/1(kR)
  [wci_vec] -> cal taui agent 3/8(wci_vec)
  [wci_vec] -> cal taui agent 4/8(wci_vec)
  [V_Phi_Reitilt_vec] -> cal taui agent 4/5(V_Phi_Reitilt_vec)
  Constant134/1 -> cal taui agent 4/1(kR)
  [dw_hat_vec] -> cal taui agent 4/6(dw_hat_vec)
  cal taui agent 4/1(tau_4) -> [tau_4]
  Constant133/1 -> cal taui agent 4/3(Ji)
  Constant135/1 -> cal taui agent 4/2(kRtilt)
  [Rei_vec] -> cal taui agent 4/7(Rei_vec)
  [dwci_vec] -> cal taui agent 4/9(dwci_vec)
  [V_Phi_Rei_vec] -> cal taui agent 4/4(V_Phi_Rei_vec)
  [wci_vec] -> cal taui agent 5/8(wci_vec)
  [dw_hat_vec] -> cal taui agent 5/6(dw_hat_vec)
  cal taui agent 5/1(tau_5) -> [tau_5]
  [V_Phi_Reitilt_vec] -> cal taui agent 5/5(V_Phi_Reitilt_vec)
  Constant137/1 -> cal taui agent 5/1(kR)
  [dwci_vec] -> cal taui agent 5/9(dwci_vec)
  Constant136/1 -> cal taui agent 5/3(Ji)
  Constant138/1 -> cal taui agent 5/2(kRtilt)
  [Rei_vec] -> cal taui agent 5/7(Rei_vec)
  [V_Phi_Rei_vec] -> cal taui agent 5/4(V_Phi_Rei_vec)
  [tau_1] -> combine tau/1(tau_1)
  [tau_2] -> combine tau/2(tau_2)
  [tau_3] -> combine tau/3(tau_3)
  [tau_4] -> combine tau/4(tau_4)
  [tau_5] -> combine tau/5(tau_5)
  combine tau/1(taui_vec) -> [taui_vec]
  [wi_vec] -> wi dynam agent 1/2(wi_vec)
  Constant175/1 -> wi dynam agent 1/1(Ji)
  [taui_vec] -> wi dynam agent 1/3(taui_vec)
  [dw_vec] -> wi dynam agent 1/4(dw_vec)
  wi dynam agent 1/1(dwi_1) -> Integrator21/1
  [taui_vec] -> wi dynam agent 2/3(taui_vec)
  [wi_vec] -> wi dynam agent 2/2(wi_vec)
  wi dynam agent 2/1(dwi_2) -> Integrator22/1
  Constant176/1 -> wi dynam agent 2/1(Ji)
  [dw_vec] -> wi dynam agent 2/4(dw_vec)
  Constant177/1 -> wi dynam agent 3/1(Ji)
  [wi_vec] -> wi dynam agent 3/2(wi_vec)
  [dw_vec] -> wi dynam agent 3/4(dw_vec)
  [taui_vec] -> wi dynam agent 3/3(taui_vec)
  wi dynam agent 3/1(dwi_3) -> Integrator23/1
  [taui_vec] -> wi dynam agent 4/3(taui_vec)
  Constant178/1 -> wi dynam agent 4/1(Ji)
  [wi_vec] -> wi dynam agent 4/2(wi_vec)
  [dw_vec] -> wi dynam agent 4/4(dw_vec)
  wi dynam agent 4/1(dwi_4) -> Integrator24/1
  [taui_vec] -> wi dynam agent 5/3(taui_vec)
  wi dynam agent 5/1(dwi_5) -> Integrator25/1
  Constant179/1 -> wi dynam agent 5/1(Ji)
  [wi_vec] -> wi dynam agent 5/2(wi_vec)
  [dw_vec] -> wi dynam agent 5/4(dw_vec)
  [wi_1] -> combine dwi/1(wi_1)
  [wi_2] -> combine dwi/2(wi_2)
  [wi_3] -> combine dwi/3(wi_3)
  [wi_4] -> combine dwi/4(wi_4)
  [wi_5] -> combine dwi/5(wi_5)
  combine dwi/1(wi_vec) -> Memory5/1
  Integrator21/1 -> [wi_1]
  Integrator22/1 -> [wi_2]
  Integrator23/1 -> [wi_3]
  Integrator24/1 -> [wi_4]
  Integrator25/1 -> [wi_5]
  [Qi_vec] -> Qi dynam agent 1/1(Qi_vec)
  [wi_vec] -> Qi dynam agent 1/2(wi_vec)
  Qi dynam agent 1/1(dQi_1) -> Integrator26/1
  Integrator26/1 -> [Qi_1]
  Qi dynam agent 2/1(dQi_2) -> Integrator27/1
  Integrator27/1 -> [Qi_2]
  [Qi_vec] -> Qi dynam agent 2/1(Qi_vec)
  [wi_vec] -> Qi dynam agent 2/2(wi_vec)
  Qi dynam agent 3/1(dQi_3) -> Integrator28/1
  [wi_vec] -> Qi dynam agent 3/2(wi_vec)
  [Qi_vec] -> Qi dynam agent 3/1(Qi_vec)
  Integrator28/1 -> [Qi_3]
  Integrator29/1 -> [Qi_4]
  [wi_vec] -> Qi dynam agent 4/2(wi_vec)
  [Qi_vec] -> Qi dynam agent 4/1(Qi_vec)
  Qi dynam agent 4/1(dQi_4) -> Integrator29/1
  Qi dynam agent 5/1(dQi_5) -> Integrator30/1
  [Qi_vec] -> Qi dynam agent 5/1(Qi_vec)
  [wi_vec] -> Qi dynam agent 5/2(wi_vec)
  Integrator30/1 -> [Qi_5]
  [Qi_1] -> combine Qi Ri/1(Qi_1)
  [Qi_2] -> combine Qi Ri/2(Qi_2)
  [Qi_3] -> combine Qi Ri/3(Qi_3)
  [Qi_4] -> combine Qi Ri/4(Qi_4)
  [Qi_5] -> combine Qi Ri/5(Qi_5)
  combine Qi Ri/1(Qi_vec) -> Memory3/1
  Constant180/1 -> cal wbarei agent 1/1(cw)
  [Reitilt_vec] -> cal wbarei agent 1/2(Reitilt_vec)
  [V_Phi_Reitilt_vec] -> cal wbarei agent 1/3(V_Phi_Reitilt_vec)
  cal wbarei agent 1/1(wbarei_1) -> [wbarei_1]
  [V_Phi_Reitilt_vec] -> cal wbarei agent 2/3(V_Phi_Reitilt_vec)
  cal wbarei agent 2/1(wbarei_2) -> [wbarei_2]
  [Reitilt_vec] -> cal wbarei agent 2/2(Reitilt_vec)
  Constant181/1 -> cal wbarei agent 2/1(cw)
  [Reitilt_vec] -> cal wbarei agent 3/2(Reitilt_vec)
  [V_Phi_Reitilt_vec] -> cal wbarei agent 3/3(V_Phi_Reitilt_vec)
  cal wbarei agent 3/1(wbarei_3) -> [wbarei_3]
  Constant182/1 -> cal wbarei agent 3/1(cw)
  [V_Phi_Reitilt_vec] -> cal wbarei agent 4/3(V_Phi_Reitilt_vec)
  [Reitilt_vec] -> cal wbarei agent 4/2(Reitilt_vec)
  cal wbarei agent 4/1(wbarei_4) -> [wbarei_4]
  Constant183/1 -> cal wbarei agent 4/1(cw)
  Constant184/1 -> cal wbarei agent 5/1(cw)
  [V_Phi_Reitilt_vec] -> cal wbarei agent 5/3(V_Phi_Reitilt_vec)
  cal wbarei agent 5/1(wbarei_5) -> [wbarei_5]
  [Reitilt_vec] -> cal wbarei agent 5/2(Reitilt_vec)
  [wbarei_5] -> combine wbarei/5(wbarei_5)
  [wbarei_4] -> combine wbarei/4(wbarei_4)
  [wbarei_1] -> combine wbarei/1(wbarei_1)
  combine wbarei/1(wbarei_vec) -> [wbarei_vec]
  [wbarei_3] -> combine wbarei/3(wbarei_3)
  [wbarei_2] -> combine wbarei/2(wbarei_2)
  [wi_vec] -> cal wei agent 1/1(wi_vec)
  [Rei_vec] -> cal wei agent 1/2(Rei_vec)
  [wci_vec] -> cal wei agent 1/3(wci_vec)
  cal wei agent 1/1(wei_1) -> [wei_1]
  [Qei_vec] -> Qei dynam agent 1/1(Qei_vec)
  [wei_vec] -> Qei dynam agent 1/2(wei_vec)
  Integrator31/1 -> [Qei_1]
  Qei dynam agent 1/1(dQei_1) -> Integrator31/1
  [Qei_vec] -> cal Rei agent 1/1(Qei_vec)
  cal Rei agent 1/1(Rei_1) -> [Rei_1]
  cal Rei agent 2/1(Rei_2) -> [Rei_2]
  cal wei agent 2/1(wei_2) -> [wei_2]
  [wei_vec] -> Qei dynam agent 2/2(wei_vec)
  [Rei_vec] -> cal wei agent 2/2(Rei_vec)
  [wi_vec] -> cal wei agent 2/1(wi_vec)
  [Qei_vec] -> Qei dynam agent 2/1(Qei_vec)
  Integrator32/1 -> [Qei_2]
  [wci_vec] -> cal wei agent 2/3(wci_vec)
  [Qei_vec] -> cal Rei agent 2/1(Qei_vec)
  Qei dynam agent 2/1(dQei_2) -> Integrator32/1
  Qei dynam agent 3/1(dQei_3) -> Integrator33/1
  [wci_vec] -> cal wei agent 3/3(wci_vec)
  [Qei_vec] -> cal Rei agent 3/1(Qei_vec)
  [wi_vec] -> cal wei agent 3/1(wi_vec)
  Integrator33/1 -> [Qei_3]
  cal wei agent 3/1(wei_3) -> [wei_3]
  [Qei_vec] -> Qei dynam agent 3/1(Qei_vec)
  cal Rei agent 3/1(Rei_3) -> [Rei_3]
  [wei_vec] -> Qei dynam agent 3/2(wei_vec)
  [Rei_vec] -> cal wei agent 3/2(Rei_vec)
  [Qei_vec] -> Qei dynam agent 4/1(Qei_vec)
  [wei_vec] -> Qei dynam agent 4/2(wei_vec)
  cal Rei agent 4/1(Rei_4) -> [Rei_4]
  Qei dynam agent 4/1(dQei_4) -> Integrator34/1
  [wi_vec] -> cal wei agent 4/1(wi_vec)
  [wci_vec] -> cal wei agent 4/3(wci_vec)
  Integrator34/1 -> [Qei_4]
  [Qei_vec] -> cal Rei agent 4/1(Qei_vec)
  [Rei_vec] -> cal wei agent 4/2(Rei_vec)
  cal wei agent 4/1(wei_4) -> [wei_4]
  [Qei_vec] -> Qei dynam agent 5/1(Qei_vec)
  [Rei_vec] -> cal wei agent 5/2(Rei_vec)
  [Qei_vec] -> cal Rei agent 5/1(Qei_vec)
  [wci_vec] -> cal wei agent 5/3(wci_vec)
  [wi_vec] -> cal wei agent 5/1(wi_vec)
  cal Rei agent 5/1(Rei_5) -> [Rei_5]
  Integrator35/1 -> [Qei_5]
  cal wei agent 5/1(wei_5) -> [wei_5]
  [wei_vec] -> Qei dynam agent 5/2(wei_vec)
  Qei dynam agent 5/1(dQei_5) -> Integrator35/1
  [wei_1] -> combine wei Qei Rei/1(wei_1)
  [wei_2] -> combine wei Qei Rei/2(wei_2)
  [wei_3] -> combine wei Qei Rei/3(wei_3)
  [wei_4] -> combine wei Qei Rei/4(wei_4)
  [wei_5] -> combine wei Qei Rei/5(wei_5)
  [Qei_1] -> combine wei Qei Rei/6(Qei_1)
  [Qei_2] -> combine wei Qei Rei/7(Qei_2)
  [Qei_3] -> combine wei Qei Rei/8(Qei_3)
  [Qei_4] -> combine wei Qei Rei/9(Qei_4)
  [Qei_5] -> combine wei Qei Rei/10(Qei_5)
  [Rei_1] -> combine wei Qei Rei/11(Rei_1)
  [Rei_2] -> combine wei Qei Rei/12(Rei_2)
  [Rei_3] -> combine wei Qei Rei/13(Rei_3)
  [Rei_4] -> combine wei Qei Rei/14(Rei_4)
  [Rei_5] -> combine wei Qei Rei/15(Rei_5)
  combine wei Qei Rei/1(wei_vec) -> Memory6/1
  combine wei Qei Rei/2(Qei_vec) -> Memory7/1
  combine wei Qei Rei/3(Rei_vec) -> Memory8/1
  cal Ri agent 1/1(Ri_1) -> [Ri_1]
  [Qi_vec] -> cal Ri agent 1/1(Qi_vec)
  cal Ri agent 2/1(Ri_2) -> [Ri_2]
  [Qi_vec] -> cal Ri agent 2/1(Qi_vec)
  [Qi_vec] -> cal Ri agent 3/1(Qi_vec)
  cal Ri agent 3/1(Ri_3) -> [Ri_3]
  [Qi_vec] -> cal Ri agent 4/1(Qi_vec)
  cal Ri agent 4/1(Ri_4) -> [Ri_4]
  cal Ri agent 5/1(Ri_5) -> [Ri_5]
  [Qi_vec] -> cal Ri agent 5/1(Qi_vec)
  [Ri_1] -> combine Qi Ri/6(Ri_1)
  [Ri_2] -> combine Qi Ri/7(Ri_2)
  [Ri_3] -> combine Qi Ri/8(Ri_3)
  [Ri_4] -> combine Qi Ri/9(Ri_4)
  [Ri_5] -> combine Qi Ri/10(Ri_5)
  combine Qi Ri/2(Ri_vec) -> Memory4/1
  [Qi_vec] -> cal Qci agent 1/1(Qi_vec)
  [Qei_vec] -> cal Qci agent 1/2(Qei_vec)
  cal Qci agent 1/1(Qci_1) -> [Qci_1]
  [Qci_1] -> cal Rci agent 1/1(Qci)
  [Qi_vec] -> cal Qci agent 2/1(Qi_vec)
  cal Qci agent 2/1(Qci_2) -> [Qci_2]
  [Qei_vec] -> cal Qci agent 2/2(Qei_vec)
  [Qi_vec] -> cal Qci agent 3/1(Qi_vec)
  [Qei_vec] -> cal Qci agent 3/2(Qei_vec)
  cal Qci agent 3/1(Qci_3) -> [Qci_3]
  cal Qci agent 4/1(Qci_4) -> [Qci_4]
  [Qei_vec] -> cal Qci agent 4/2(Qei_vec)
  [Qi_vec] -> cal Qci agent 4/1(Qi_vec)
  [Qi_vec] -> cal Qci agent 5/1(Qi_vec)
  [Qei_vec] -> cal Qci agent 5/2(Qei_vec)
  cal Qci agent 5/1(Qci_5) -> [Qci_5]
  [Qci_5] -> combine Qci Rci/5(Qci_5)
  [Qci_4] -> combine Qci Rci/4(Qci_4)
  [Rci_3] -> combine Qci Rci/8(Rci_3)
  [Qci_1] -> combine Qci Rci/1(Qci_1)
  [Rci_5] -> combine Qci Rci/10(Rci_5)
  [Qci_3] -> combine Qci Rci/3(Qci_3)
  combine Qci Rci/1(Qci_vec) -> Memory16/1
  combine Qci Rci/2(Rci_vec) -> Memory17/1
  [Qci_2] -> combine Qci Rci/2(Qci_2)
  [Rci_2] -> combine Qci Rci/7(Rci_2)
  [Rci_4] -> combine Qci Rci/9(Rci_4)
  [Rci_1] -> combine Qci Rci/6(Rci_1)
  cal Reitilt agent 1/1(Reitilt_1) -> [Reitilt_1]
  cal weitilt agent 1/1(weitilt_1) -> [weitilt_1]
  [weitilt_vec] -> Qeitilt dynam agent 1/2(weitilt_vec)
  [Reitilt_vec] -> cal weitilt agent 1/2(Reitilt_vec)
  [wei_vec] -> cal weitilt agent 1/1(wei_vec)
  [Qeitilt_vec] -> Qeitilt dynam agent 1/1(Qeitilt_vec)
  Integrator36/1 -> [Qeitilt_1]
  [wbarei_vec] -> cal weitilt agent 1/3(wbarei_vec)
  [Qeitilt_vec] -> cal Reitilt agent 1/1(Qeitilt_vec)
  Qeitilt dynam agent 1/1(dQeitilt_1) -> Integrator36/1
  Integrator37/1 -> [Qeitilt_2]
  [Qeitilt_vec] -> cal Reitilt agent 2/1(Qeitilt_vec)
  [Reitilt_vec] -> cal weitilt agent 2/2(Reitilt_vec)
  [wbarei_vec] -> cal weitilt agent 2/3(wbarei_vec)
  [weitilt_vec] -> Qeitilt dynam agent 2/2(weitilt_vec)
  [Qeitilt_vec] -> Qeitilt dynam agent 2/1(Qeitilt_vec)
  cal Reitilt agent 2/1(Reitilt_2) -> [Reitilt_2]
  cal weitilt agent 2/1(weitilt_2) -> [weitilt_2]
  Qeitilt dynam agent 2/1(dQeitilt_2) -> Integrator37/1
  [wei_vec] -> cal weitilt agent 2/1(wei_vec)
  cal weitilt agent 3/1(weitilt_3) -> [weitilt_3]
  cal Reitilt agent 3/1(Reitilt_3) -> [Reitilt_3]
  [weitilt_vec] -> Qeitilt dynam agent 3/2(weitilt_vec)
  [wbarei_vec] -> cal weitilt agent 3/3(wbarei_vec)
  Qeitilt dynam agent 3/1(dQeitilt_3) -> Integrator38/1
  [Reitilt_vec] -> cal weitilt agent 3/2(Reitilt_vec)
  [Qeitilt_vec] -> Qeitilt dynam agent 3/1(Qeitilt_vec)
  [wei_vec] -> cal weitilt agent 3/1(wei_vec)
  [Qeitilt_vec] -> cal Reitilt agent 3/1(Qeitilt_vec)
  Integrator38/1 -> [Qeitilt_3]
  [Qeitilt_vec] -> Qeitilt dynam agent 4/1(Qeitilt_vec)
  Qeitilt dynam agent 4/1(dQeitilt_4) -> Integrator39/1
  [Qeitilt_vec] -> cal Reitilt agent 4/1(Qeitilt_vec)
  [weitilt_vec] -> Qeitilt dynam agent 4/2(weitilt_vec)
  Integrator39/1 -> [Qeitilt_4]
  cal Reitilt agent 4/1(Reitilt_4) -> [Reitilt_4]
  [Reitilt_vec] -> cal weitilt agent 4/2(Reitilt_vec)
  [wei_vec] -> cal weitilt agent 4/1(wei_vec)
  cal weitilt agent 4/1(weitilt_4) -> [weitilt_4]
  [wbarei_vec] -> cal weitilt agent 4/3(wbarei_vec)
  [weitilt_vec] -> Qeitilt dynam agent 5/2(weitilt_vec)
  cal weitilt agent 5/1(weitilt_5) -> [weitilt_5]
  [wei_vec] -> cal weitilt agent 5/1(wei_vec)
  cal Reitilt agent 5/1(Reitilt_5) -> [Reitilt_5]
  [wbarei_vec] -> cal weitilt agent 5/3(wbarei_vec)
  Qeitilt dynam agent 5/1(dQeitilt_5) -> Integrator40/1
  [Qeitilt_vec] -> Qeitilt dynam agent 5/1(Qeitilt_vec)
  Integrator40/1 -> [Qeitilt_5]
  [Qeitilt_vec] -> cal Reitilt agent 5/1(Qeitilt_vec)
  [Reitilt_vec] -> cal weitilt agent 5/2(Reitilt_vec)
  [Reitilt_1] -> combine weitilt Qeitilt Reitilt/11(Reitilt_1)
  [Qeitilt_3] -> combine weitilt Qeitilt Reitilt/8(Qeitilt_3)
  [weitilt_1] -> combine weitilt Qeitilt Reitilt/1(weitilt_1)
  [Reitilt_2] -> combine weitilt Qeitilt Reitilt/12(Reitilt_2)
  [Qeitilt_4] -> combine weitilt Qeitilt Reitilt/9(Qeitilt_4)
  [Reitilt_5] -> combine weitilt Qeitilt Reitilt/15(Reitilt_5)
  [Reitilt_3] -> combine weitilt Qeitilt Reitilt/13(Reitilt_3)
  combine weitilt Qeitilt Reitilt/1(weitilt_vec) -> Memory9/1
  [weitilt_3] -> combine weitilt Qeitilt Reitilt/3(weitilt_3)
  combine weitilt Qeitilt Reitilt/3(Reitilt_vec) -> Memory11/1
  [weitilt_2] -> combine weitilt Qeitilt Reitilt/2(weitilt_2)
  [weitilt_5] -> combine weitilt Qeitilt Reitilt/5(weitilt_5)
  [Qeitilt_5] -> combine weitilt Qeitilt Reitilt/10(Qeitilt_5)
  [Qeitilt_1] -> combine weitilt Qeitilt Reitilt/6(Qeitilt_1)
  [Reitilt_4] -> combine weitilt Qeitilt Reitilt/14(Reitilt_4)
  combine weitilt Qeitilt Reitilt/2(Qeitilt_vec) -> Memory10/1
  [Qeitilt_2] -> combine weitilt Qeitilt Reitilt/7(Qeitilt_2)
  [weitilt_4] -> combine weitilt Qeitilt Reitilt/4(weitilt_4)
  [V_Phi_Rei_vec] -> To Workspace1/1
  [V_Phi_Reitilt_vec] -> To Workspace6/1
  [Qeitilt_vec] -> To Workspace7/1
  [Qei_vec] -> depart Qe3/1(x), depart Qe5/1(x), depart Qe4/1(x), depart Qe2/1(x), depart Qe1/1(x)
  depart Qe1/1(y) -> Display38/1, Demux33/1
  Demux33/1 -> Scope/1
  Demux33/2 -> Scope/2
  Demux33/3 -> Scope/3
  Demux33/4 -> Scope/4
  Demux34/1 -> Scope3/1
  Demux34/3 -> Scope3/3
  Demux34/2 -> Scope3/2
  Demux34/4 -> Scope3/4
  depart Qe2/1(y) -> Display42/1, Demux34/1
  Demux35/1 -> Scope4/1
  Demux35/3 -> Scope4/3
  Demux35/2 -> Scope4/2
  Demux35/4 -> Scope4/4
  depart Qe3/1(y) -> Display43/1, Demux35/1
  Demux36/1 -> Scope5/1
  Demux36/3 -> Scope5/3
  Demux36/2 -> Scope5/2
  Demux36/4 -> Scope5/4
  depart Qe4/1(y) -> Display59/1, Demux36/1
  Demux37/1 -> Scope6/1
  Demux37/3 -> Scope6/3
  Demux37/2 -> Scope6/2
  Demux37/4 -> Scope6/4
  depart Qe5/1(y) -> Display60/1, Demux37/1
  Demux57/1 -> Scope7/1
  Demux60/4 -> Scope10/4
  Demux60/1 -> Scope10/1
  Demux60/3 -> Scope10/3
  Demux58/4 -> Scope8/4
  depart Qe5tilt/1(y) -> Display65/1, Demux61/1
  depart Qe3tilt/1(y) -> Display63/1, Demux59/1
  [Qeitilt_vec] -> depart Qe3tilt/1(x), depart Qe5tilt/1(x), depart Qe4tilt/1(x), depart Qe2tilt/1(x), depart Qe1tilt/1(x)
  Demux61/2 -> Scope11/2
  Demux61/3 -> Scope11/3
  Demux61/1 -> Scope11/1
  Demux60/2 -> Scope10/2
  Demux57/2 -> Scope7/2
  Demux57/4 -> Scope7/4
  depart Qe4tilt/1(y) -> Display64/1, Demux60/1
  Demux58/3 -> Scope8/3
  depart Qe2tilt/1(y) -> Display62/1, Demux58/1
  Demux58/1 -> Scope8/1
  Demux61/4 -> Scope11/4
  Demux57/3 -> Scope7/3
  Demux59/4 -> Scope9/4
  Demux58/2 -> Scope8/2
  Demux59/2 -> Scope9/2
  Demux59/3 -> Scope9/3
  Demux59/1 -> Scope9/1
  depart Qe1tilt/1(y) -> Display61/1, Demux57/1
  Demux62/1 -> Scope17/1
  depart we5/1(y) -> Display70/1, Demux66/1
  Demux65/3 -> Scope12/3
  Demux65/2 -> Scope12/2
  Demux66/3 -> Scope16/3
  Demux66/2 -> Scope16/2
  Demux66/1 -> Scope16/1
  Demux65/1 -> Scope12/1
  [wei_vec] -> depart we3/1(x), depart we5/1(x), depart we4/1(x), depart we2/1(x), depart we1/1(x)
  depart we3/1(y) -> Display68/1, Demux64/1
  Demux63/1 -> Scope18/1
  depart we2/1(y) -> Display67/1, Demux63/1
  Demux63/3 -> Scope18/3
  depart we4/1(y) -> Display69/1, Demux65/1
  Demux62/3 -> Scope17/3
  Demux64/1 -> Scope19/1
  Demux64/3 -> Scope19/3
  Demux63/2 -> Scope18/2
  depart we1/1(y) -> Display66/1, Demux62/1
  Demux64/2 -> Scope19/2
  Demux62/2 -> Scope17/2
  Demux70/3 -> Scope20/3
  [weitilt_vec] -> depart we3tilt/1(x), depart we5tilt/1(x), depart we4tilt/1(x), depart we2tilt/1(x), depart we1tilt/1(x)
  depart we4tilt/1(y) -> Display74/1, Demux70/1
  Demux67/3 -> Scope22/3
  Demux68/2 -> Scope23/2
  Demux69/3 -> Scope24/3
  Demux69/1 -> Scope24/1
  depart we2tilt/1(y) -> Display72/1, Demux68/1
  depart we5tilt/1(y) -> Display75/1, Demux71/1
  Demux68/1 -> Scope23/1
  depart we3tilt/1(y) -> Display73/1, Demux69/1
  Demux68/3 -> Scope23/3
  Demux69/2 -> Scope24/2
  depart we1tilt/1(y) -> Display71/1, Demux67/1
  Demux67/2 -> Scope22/2
  Demux70/1 -> Scope20/1
  Demux70/2 -> Scope20/2
  Demux67/1 -> Scope22/1
  Demux71/1 -> Scope21/1
  Demux71/3 -> Scope21/3
  Demux71/2 -> Scope21/2
  Demux75/3 -> Scope25/3
  [V_Phi_Rei_vec] -> depart V_Phi_Re3/1(x), depart V_Phi_Re5/1(x), depart V_Phi_Re4/1(x), depart V_Phi_Re2/1(x), depart V_Phi_Re1/1(x)
  depart V_Phi_Re4/1(y) -> Display79/1, Demux75/1
  Demux72/3 -> Scope27/3
  Demux73/2 -> Scope28/2
  Demux74/3 -> Scope29/3
  Demux74/1 -> Scope29/1
  depart V_Phi_Re2/1(y) -> Display77/1, Demux73/1
  depart V_Phi_Re5/1(y) -> Display80/1, Demux76/1
  Demux73/1 -> Scope28/1
  depart V_Phi_Re3/1(y) -> Display78/1, Demux74/1
  Demux73/3 -> Scope28/3
  Demux74/2 -> Scope29/2
  depart V_Phi_Re1/1(y) -> Display76/1, Demux72/1
  Demux72/2 -> Scope27/2
  Demux75/1 -> Scope25/1
  Demux75/2 -> Scope25/2
  Demux72/1 -> Scope27/1
  Demux76/1 -> Scope26/1
  Demux76/3 -> Scope26/3
  Demux76/2 -> Scope26/2
  depart V_Phi_Re2tilt/1(y) -> Display82/1, Demux78/1
  depart V_Phi_Re5tilt/1(y) -> Display85/1, Demux81/1
  Demux79/3 -> Scope34/3
  Demux78/2 -> Scope33/2
  Demux77/3 -> Scope32/3
  depart V_Phi_Re4tilt/1(y) -> Display84/1, Demux80/1
  [V_Phi_Reitilt_vec] -> depart V_Phi_Re3tilt/1(x), depart V_Phi_Re5tilt/1(x), depart V_Phi_Re4tilt/1(x), depart V_Phi_Re2tilt/1(x), depart V_Phi_Re1tilt/1(x)
  Demux80/3 -> Scope30/3
  Demux77/2 -> Scope32/2
  Demux80/1 -> Scope30/1
  depart V_Phi_Re1tilt/1(y) -> Display81/1, Demux77/1
  Demux78/1 -> Scope33/1
  Demux79/1 -> Scope34/1
  Demux79/2 -> Scope34/2
  Demux77/1 -> Scope32/1
  Demux78/3 -> Scope33/3
  Demux81/2 -> Scope31/2
  Demux81/3 -> Scope31/3
  Demux81/1 -> Scope31/1
  Demux80/2 -> Scope30/2
  depart V_Phi_Re3tilt/1(y) -> Display83/1, Demux79/1
  [dw_vec] -> depart dw1 dw_hat_1/1(x1)
  [dw_hat_vec] -> depart dw1 dw_hat_1/2(x2)
  depart dw1 dw_hat_1/1(y1) -> Display86/1, Demux82/1
  Mux/1 -> Scope35/1
  Mux56/1 -> Scope35/2
  Mux57/1 -> Scope35/3
  depart dw1 dw_hat_1/2(y2) -> Display87/1, Demux83/1
  Demux82/1 -> Mux/1
  Demux83/1 -> Mux/2
  Demux82/2 -> Mux56/1
  Demux82/3 -> Mux57/1
  Demux83/2 -> Mux56/2
  Demux83/3 -> Mux57/2
  Demux85/1 -> Mux58/2
  Mux60/1 -> Scope36/3
  Demux84/1 -> Mux58/1
  depart dw2 dw_hat_2/1(y1) -> Display88/1, Demux84/1
  Demux85/2 -> Mux59/2
  Demux84/3 -> Mux60/1
  depart dw2 dw_hat_2/2(y2) -> Display89/1, Demux85/1
  Mux59/1 -> Scope36/2
  Demux84/2 -> Mux59/1
  Demux85/3 -> Mux60/2
  Mux58/1 -> Scope36/1
  [dw_vec] -> depart dw2 dw_hat_2/1(x1)
  [dw_hat_vec] -> depart dw2 dw_hat_2/2(x2)
  [dw_vec] -> depart dw3 dw_hat_3/1(x1)
  [dw_hat_vec] -> depart dw3 dw_hat_3/2(x2)
  Mux61/1 -> Scope37/1
  depart dw3 dw_hat_3/1(y1) -> Display90/1, Demux86/1
  Demux86/3 -> Mux63/1
  Demux87/3 -> Mux63/2
  Mux62/1 -> Scope37/2
  Demux86/2 -> Mux62/1
  Demux87/2 -> Mux62/2
  Demux86/1 -> Mux61/1
  Demux87/1 -> Mux61/2
  Mux63/1 -> Scope37/3
  depart dw3 dw_hat_3/2(y2) -> Display91/1, Demux87/1
  [dw_vec] -> depart dw4 dw_hat_4/1(x1)
  [dw_hat_vec] -> depart dw4 dw_hat_4/2(x2)
  Demux89/1 -> Mux64/2
  Mux66/1 -> Scope38/3
  Demux88/1 -> Mux64/1
  depart dw4 dw_hat_4/1(y1) -> Display92/1, Demux88/1
  Demux89/2 -> Mux65/2
  Demux88/3 -> Mux66/1
  depart dw4 dw_hat_4/2(y2) -> Display93/1, Demux89/1
  Mux65/1 -> Scope38/2
  Demux88/2 -> Mux65/1
  Demux89/3 -> Mux66/2
  Mux64/1 -> Scope38/1
  [dw_vec] -> depart dw4 dw_hat_1/1(x1)
  [dw_hat_vec] -> depart dw4 dw_hat_1/2(x2)
  Demux90/3 -> Mux69/1
  Demux90/1 -> Mux67/1
  Demux91/1 -> Mux67/2
  Mux69/1 -> Scope39/3
  Demux90/2 -> Mux68/1
  Mux68/1 -> Scope39/2
  Demux91/3 -> Mux69/2
  Demux91/2 -> Mux68/2
  depart dw4 dw_hat_1/1(y1) -> Display94/1, Demux90/1
  Mux67/1 -> Scope39/1
  depart dw4 dw_hat_1/2(y2) -> Display95/1, Demux91/1
  Memory3/1 -> [Qi_vec]
  Memory4/1 -> [Ri_vec]
  Memory5/1 -> [wi_vec]
  Memory6/1 -> [wei_vec]
  Memory7/1 -> [Qei_vec]
  Memory8/1 -> [Rei_vec]
  Memory9/1 -> [weitilt_vec]
  Memory10/1 -> [Qeitilt_vec]
  Memory11/1 -> [Reitilt_vec]
  Memory14/1 -> Display100/1, [wci_vec]
  Memory15/1 -> Display101/1, [dwci_vec]
  Memory16/1 -> [Qci_vec]
  Memory17/1 -> [Rci_vec]
  cal Rci agent 1/1(Rci_1) -> [Rci_1]
  cal Rci agent 2/1(Rci_2) -> [Rci_2]
  [Qci_2] -> cal Rci agent 2/1(Qci)
  [Qci_3] -> cal Rci agent 3/1(Qci)
  cal Rci agent 3/1(Rci_3) -> [Rci_3]
  cal Rci agent 4/1(Rci_4) -> [Rci_4]
  [Qci_4] -> cal Rci agent 4/1(Qci)
  [Qci_5] -> cal Rci agent 5/1(Qci_vec)
  cal Rci agent 5/1(Rci_5) -> [Rci_5]
  Demux101/4 -> Scope49/4
  depart wc3/1(y) -> Display99/1, Demux94/1
  Demux97/3 -> Scope45/3
  Demux100/2 -> Scope48/2
  Demux94/1 -> Scope42/1
  Demux100/4 -> Scope48/4
  Demux97/1 -> Scope45/1
  Demux99/4 -> Scope47/4
  Demux97/2 -> Scope45/2
  Demux92/3 -> Scope40/3
  Demux92/2 -> Scope40/2
  Demux98/4 -> Scope46/4
  Demux100/1 -> Scope48/1
  Demux96/3 -> Scope44/3
  depart Qc4/1(y) -> Display107/1, Demux100/1
  Demux101/1 -> Scope49/1
  Demux100/3 -> Scope48/3
  Demux93/3 -> Scope41/3
  depart wc5/1(y) -> Display103/1, Demux96/1
  Demux96/1 -> Scope44/1
  Demux96/2 -> Scope44/2
  Demux98/3 -> Scope46/3
  Demux101/2 -> Scope49/2
  depart wc2/1(y) -> Display98/1, Demux93/1
  Demux97/4 -> Scope45/4
  Demux98/2 -> Scope46/2
  Demux101/3 -> Scope49/3
  Demux94/3 -> Scope42/3
  depart Qc3/1(y) -> Display106/1, Demux99/1
  Demux94/2 -> Scope42/2
  Demux95/2 -> Scope43/2
  Demux99/2 -> Scope47/2
  depart Qc2/1(y) -> Display105/1, Demux98/1
  Demux98/1 -> Scope46/1
  [Qci_vec] -> depart Qc3/1(x), depart Qc5/1(x), depart Qc4/1(x), depart Qc2/1(x), depart Qc1/1(x)
  depart Qc5/1(y) -> Display97/1, Demux101/1
  depart wc4/1(y) -> Display102/1, Demux95/1
  [wci_vec] -> depart wc3/1(x), depart wc5/1(x), depart wc4/1(x), depart wc2/1(x), depart wc1/1(x)
  Demux93/2 -> Scope41/2
  Demux92/1 -> Scope40/1
  Demux95/3 -> Scope43/3
  depart Qc1/1(y) -> Display104/1, Demux97/1
  Demux99/1 -> Scope47/1
  depart wc1/1(y) -> Display96/1, Demux92/1
  Demux93/1 -> Scope41/1
  Demux95/1 -> Scope43/1
  Demux99/3 -> Scope47/3
  [weitilt_5] -> Integrator50/1
  [weitilt_1] -> Integrator41/1
  Integrator45/1 -> [V_Phi_Rei_1]
  [weitilt_4] -> Integrator48/1
  [wei_3] -> Integrator44/1
  combine Qci Rci1/2(V_Phi_Reitilt_vec) -> Memory13/1
  [wei_1] -> Integrator45/1
  [wei_2] -> Integrator42/1
  [V_Phi_Reitilt_1] -> combine Qci Rci1/6(V_Phi_Reitilt_1)
  [V_Phi_Rei_3] -> combine Qci Rci1/3(V_Phi_Rei_3)
  Integrator42/1 -> [V_Phi_Rei_2]
  Integrator44/1 -> [V_Phi_Rei_3]
  [wei_4] -> Integrator47/1
  Integrator49/1 -> [V_Phi_Rei_5]
  Integrator48/1 -> [V_Phi_Reitilt_4]
  [wei_5] -> Integrator49/1
  [V_Phi_Reitilt_2] -> combine Qci Rci1/7(V_Phi_Reitilt_2)
  Memory13/1 -> [V_Phi_Reitilt_vec]
  [V_Phi_Reitilt_4] -> combine Qci Rci1/9(V_Phi_Reitilt_4)
  [weitilt_2] -> Integrator43/1
  Integrator50/1 -> [V_Phi_Reitilt_5]
  Memory12/1 -> [V_Phi_Rei_vec]
  [V_Phi_Rei_2] -> combine Qci Rci1/2(V_Phi_Rei_2)
  [V_Phi_Rei_5] -> combine Qci Rci1/5(V_Phi_Rei_5)
  Integrator47/1 -> [V_Phi_Rei_4]
  [V_Phi_Reitilt_3] -> combine Qci Rci1/8(V_Phi_Reitilt_3)
  combine Qci Rci1/1(V_Phi_Rei_vec) -> Memory12/1
  [weitilt_3] -> Integrator46/1
  [V_Phi_Rei_1] -> combine Qci Rci1/1(V_Phi_Rei_1)
  [V_Phi_Reitilt_5] -> combine Qci Rci1/10(V_Phi_Reitilt_5)
  Integrator41/1 -> [V_Phi_Reitilt_1]
  [V_Phi_Rei_4] -> combine Qci Rci1/4(V_Phi_Rei_4)
  Integrator43/1 -> [V_Phi_Reitilt_2]
  Integrator46/1 -> [V_Phi_Reitilt_3]
  [dw_vec] -> To Workspace8/1
  [dw_hat_vec] -> To Workspace9/1
  cal error dw_tilt/1(dw_tilt_vec) -> [dw_tilt_vec]
  [dw_vec] -> cal error dw_tilt/1(dw_vec)
  [dw_hat_vec] -> cal error dw_tilt/2(dw_hat_vec)
  [dw_tilt_vec] -> To Workspace10/1
  [sigma_bar_w_hat_vec] -> To Workspace12/1
  [sigma_w_vec] -> To Workspace14/1
  [sigma_bar_w_vec] -> To Workspace15/1
  [tsim] -> process velocity/11(t)
  Constant199/1 -> process velocity/2(T1)
  Step/1 -> leader eta0 Integrator/2
  leader eta0 Integrator/1 -> [eta0], leader ksi0 Integrator/1
  Constant185/1 -> leader control input/2(T1)
  [u0] -> leader eta0 Integrator/1
  Constant187/1 -> process velocity/7(R1)
  [V_init_out] -> leader eta0 Integrator/3
  [u0] -> control input generator agent 5/1(u0)
  [u0] -> control input generator agent 1/1(u0)
  [ui_n_5] -> combine norminal formation control input/5(ui_5)
  [ui_n_3] -> combine norminal formation control input/3(ui_3)
  Constant195/1 -> leader control input/6(Rx2)
  Memory/1 -> [ui_vec]
  [ui_n_4] -> combine norminal formation control input/4(ui_4)
  Clock/1 -> [tsim]
  [u0] -> control input generator agent 3/1(u0)
  control input generator agent 1/1(ui) -> [ui_n_1]
  control input generator agent 2/1(ui) -> [ui_n_2]
  [ui_n_2] -> combine norminal formation control input/2(ui_2)
  [ui_n_1] -> combine norminal formation control input/1(ui_1)
  control input generator agent 4/1(ui) -> [ui_n_4]
  control input generator agent 3/1(ui) -> [ui_n_3]
  [u0] -> control input generator agent 2/1(u0)
  process velocity/1(V_init_out) -> [V_init_out]
  Constant200/1 -> process velocity/4(PZ0)
  Demux1/1 -> ksi_0/1
  Constant192/1 -> leader control input/3(T2)
  Demux1/2 -> ksi_0/2
  combine norminal formation control input/1(ui_vec) -> Memory/1
  Demux22/3 -> eta_0/3
  [tsim] -> leader control input/1(t)
  control input generator agent 5/1(ui) -> [ui_n_5]
  Constant190/1 -> process velocity/9(Ry2)
  Constant198/1 -> process velocity/3(T2)
  leader ksi0 Integrator/1 -> [ksi0]
  Constant191/1 -> process velocity/8(Rx2)
  [u0] -> control input generator agent 4/1(u0)
  Demux1/3 -> ksi_0/3
  Constant189/1 -> process velocity/10(Rz2)
  Demux22/2 -> eta_0/2
  Constant201/1 -> process velocity/5(PZ1)
  Constant194/1 -> leader control input/5(R1)
  Constant196/1 -> leader control input/7(Ry2)
  Demux22/1 -> eta_0/1
  [ksi0] -> Demux1/1
  Constant193/1 -> leader control input/4(R0)
  Constant186/1 -> process velocity/6(R0)
  [eta0] -> Demux22/1
  Constant197/1 -> leader control input/8(Rz2)
  Constant188/1 -> process velocity/1(T0)
  leader control input/1(u0) -> [u0]
  generate angular rate disturbance agent 5/1(dw_5) -> [dw_5]
  [dw_2] -> combine tau1/2(dw_2)
  Constant561/1 -> generate angular rate disturbance agent 2/1(dw_aa_t)
  Constant558/1 -> generate angular rate disturbance agent 1/2(dw_ff_t)
  Constant559/1 -> generate angular rate disturbance agent 1/3(dw_phi_t)
  Constant563/1 -> generate angular rate disturbance agent 2/3(dw_phi_t)
  Constant566/1 -> generate angular rate disturbance agent 3/3(dw_phi_t)
  [tsim] -> generate angular rate disturbance agent 4/4(t)
  [tsim] -> generate angular rate disturbance agent 2/4(t)
  [dw_5] -> combine tau1/5(dw_5)
  Constant562/1 -> generate angular rate disturbance agent 2/2(dw_ff_t)
  [tsim] -> generate angular rate disturbance agent 3/4(t)
  Constant565/1 -> generate angular rate disturbance agent 3/2(dw_ff_t)
  generate angular rate disturbance agent 3/1(dw_3) -> [dw_3]
  Constant572/1 -> generate angular rate disturbance agent 5/2(dw_ff_t)
  [dw_4] -> combine tau1/4(dw_4)
  Constant557/1 -> generate angular rate disturbance agent 1/1(dw_aa_t)
  Constant569/1 -> generate angular rate disturbance agent 4/3(dw_phi_t)
  Constant568/1 -> generate angular rate disturbance agent 4/2(dw_ff_t)
  Constant564/1 -> generate angular rate disturbance agent 3/1(dw_aa_t)
  generate angular rate disturbance agent 4/1(dw_4) -> [dw_4]
  generate angular rate disturbance agent 1/1(dw_1) -> [dw_1]
  Constant573/1 -> generate angular rate disturbance agent 5/3(dw_phi_t)
  [tsim] -> generate angular rate disturbance agent 5/4(t)
  Constant567/1 -> generate angular rate disturbance agent 4/1(dw_aa_t)
  Constant570/1 -> generate angular rate disturbance agent 5/1(dw_aa_t)
  [dw_1] -> combine tau1/1(dw_1)
  [tsim] -> generate angular rate disturbance agent 1/4(t)
  [dw_3] -> combine tau1/3(dw_3)
  generate angular rate disturbance agent 2/1(dw_2) -> [dw_2]
  combine tau1/1(dw_vec) -> [dw_vec]
